simulink library "DAEMOT_Lib"  (R2019b)
settings: Solver=ode45  StartTime=0.0  StopTime=10.0  FixedStep=0.1  RelTol=1e-3
undefined symbols (not defined in the file or in its folder): Controller, CP, Ctrl, Ctrl_Fcn, Elec1, f, F2, Fluid, lag1, Mission, Moody, PropellerProp, rev_comms_sink
libraries: $bdroot x200, instrumentlib x21, simulink x5, dspsigops x2
(part 4 of 13)

== system DAEMOT_Lib/Support Functions ==
  Data Manager : Subsystem  mask{null=0}
      mask init:
      | set_param(gcb, 'LinkStatus', 'inactive')    % disable the library link
      settings: OpenFcn=data_manager
      mask Display: str ='Data Manager\n(Double click to select variables for output)'; fprintf(str)
  Data_Sink : Subsystem  LoadFcn=|  InitFcn=|  mask(Data Sink){}
      LoadFcn=|
      | h      = get_param(gcb,'handle');   % Get block handle                           
      | hblock = get(h);     % Parse out handles structure
      | 
      | str = [hblock.Path(numel(bdroot)+2:end), hblock.Name];
      | str(~ismember(str,['A':'Z' 'a':'z' '0':'9' '_'])) = '';                     
      | set_param([gcb, '/global_data_goto'],'GotoTag',['gdata_',str]);
      |                                
      |                                                                                  
      | clear h hblock str
      InitFcn=|
      | h      = get_param(gcb,'handle');   % Get block handle                           
      | hblock = get(h);     % Parse out handles structure
      | 
      | str = [hblock.Path(numel(bdroot)+2:end), hblock.Name];
      | str(~ismember(str,['A':'Z' 'a':'z' '0':'9' '_'])) = '';                     
      | set_param([gcb, '/global_data_goto'],'GotoTag',['gdata_',str]);
      |                                
      |                                                                                  
      | clear h hblock str
      mask help:
      | Input to this block should be a bus signal with named signals.
      |
      | Bus signals sent to this block will be read by the Data Manager.
      | The Data Manager will handle the global routing of signals.
      |
      | This block should be placed under the mask of components.
      settings: CopyFcn=|
      | h      = get_param(gcb,'handle');   % Get block handle
      | hblock = get(h);     % Parse out handles structure
      | 
      | str = [hblock.Path(numel(bdroot)+2:end), hblock.Name];
      | str(~ismember(str,['A':'Z' 'a':'z' '0':'9' '_'])) = '';
      | set_param([gcb, '/global_data_goto'],'GotoTag',['gdata_',str]);
      | 
      | 
      | clear h hblock str
      settings: NameChangeFcn=|
      | h      = get_param(gcb,'handle');   % Get block handle
      | hblock = get(h);     % Parse out handles structure
      | 
      | str = [hblock.Path(numel(bdroot)+2:end), hblock.Name];
      | str(~ismember(str,['A':'Z' 'a':'z' '0':'9' '_'])) = '';
      | set_param([gcb, '/global_data_goto'],'GotoTag',['gdata_',str]);
      | 
      | 
      | clear h hblock str
      mask Display: text(0.25,0.5,'Data Sink')
  Generic Graph Model : Subsystem  mask{G_NAME=Elec1, MODE=DAE Graph}
      mask prompts: G_NAME "Graph Name"; MODE "Graph Type"
      mask init:
      | %%%%% update the variant subsystem %%%%%%%%%%%%%
      | simulationStatus =  get_param(bdroot,'SimulationStatus');
      | choice = get_param(gcb,'MODE');
      | vssBlk = [gcb, '/Variant Subsystem'];
      | oldVariant = get_param(gcb,'OverrideUsingVariant');
      | if strcmp(choice,'Dynamic Graph')   
      |     set_param(vssBlk, 'OverrideUsingVariant', 'Dynamic_Graph');
      | else  
      |     set_param(vssBlk, 'OverrideUsingVariant', 'DAE_Graph');
      | end
      | 
      | %%%%%%% load in graph for property lookups %%%%%%%%%
      | GRAPH_NAME = get_param(gcb,'G_NAME');
      | 
      | Graph = evalin('base',GRAPH_NAME);
      | 
      | h      = get_param(gcb,'handle');   % Get block handle
      | blk    = gcb;
      | hblock = get(h);     % Parse out handles structure
      | 
      | blk = [gcb,'/Variant Subsystem/',choice]; 
      | 
      | if Graph.Nu == 0
      |     Nu = 1;
      | else
      |     Nu = Graph.Nu;
      | end
      | 
      | if Graph.Nsv == 0
      |     Nsv = 1;
      | else
      |     Nsv = Graph.Nsv;
      | end
      | 
      | %%%%%%%%% 1D Property Lookups %%%%%%%%%%%%%%%%%%%%%%%%%%%%%%%%%%%%
      | % delete extra blocks
      | temp = get_param([blk,'/mux_1D'],'Inputs');
      | try % check if previous operation had zero 1-D lookups
      |     get_param([blk,'/map_1D_1'],'Table');
      |     flag = 1; %if we find a lookup table, set flag high
      | catch
      |     flag = 0; %if previous operation had zero 1-D lookups, set flag low
      | end
      | 
      | if Graph.ND1_map == 0 %if there are zero property lookups, make sure the mux is of size 1
      |     set_param([blk,'/mux_1D'],'Inputs','1')
      | else
      |     set_param([blk,'/mux_1D'],'Inputs',num2str(Graph.ND1_map))
      | end
      | % delete extra blocks and lines
      | for i = Graph.ND1_map+1:str2num(temp)
      |     try
      |         delete_block([blk,'/select_1D_',num2str(i)])
      |         delete_block([blk,'/map_1D_',num2str(i)])
      |         delete_block([blk,'/mod_1D_',num2str(i)])
      |         delete_unconnected_lines(blk)
      |     catch
      |     end
      | end
      | 
      | if flag == 0 %modifier to make sure 1st lookup is added if previous graph had zero lookups
      |     temp = num2str((str2num(temp)-1));
      | end
      | 
      | %re-label existing blocks
      | if Graph.ND1_map ~= 0
      |     for i = 1:str2num(temp)     
      |         set_param([blk,'/select_1D_',num2str(i)],'InputPortWidth',[GRAPH_NAME,'.Nv+',num2str(Nsv),'+',num2str(Nu)])
      |         if Graph.Props.D1_map{2,i} == 2
      |             set_param([blk,'/select_1D_',num2str(i)],'Indices',char(horzcat(GRAPH_NAME,'.Nv+',num2str(Nsv),'+Elec.Props.D1_map{1,',num2str(i),'}')))
      |         else
      |             set_param([blk,'/select_1D_',num2str(i)],'Indices',char(horzcat(GRAPH_NAME,'.Props.D1_map{1,',num2str(i),'}')))
      |         end
      |         set_param([blk,'/map_1D_',num2str(i)],'BreakpointsForDimension1',char(horzcat(GRAPH_NAME,'.Props.D1_map{3,',num2str(i),'}')))
      |         set_param([blk,'/map_1D_',num2str(i)],'Table',char(horzcat(GRAPH_NAME,'.Props.D1_map{4,',num2str(i),'}')))
      |         if Graph.Props.D1_map{6,i} == 2
      |             set_param([blk,'/mod_1D_',num2str(i)],'Operator','reciprocal')
      |         else
      |             set_param([blk,'/mod_1D_',num2str(i)],'Operator','transpose')
      |         end
      |     end
      | end
      | 
      | 
      | % add blocks
      | if Graph.ND1_map ~= 0
      |     for i = str2num(temp)+1:Graph.ND1_map
      |         add_block('simulink/Signal Routing/Selector',        [blk,'/select_1D_',num2str(i)],    'Position',[1355 16+i*80 1355+40 16+i*80+38]);
      |         add_block('simulink/Lookup Tables/1-D Lookup Table', [blk,'/map_1D_',num2str(i)],    'Position',[1435 3+i*80 1435+65 3+i*80+64]);
      |         add_block('simulink/Math Operations/Math Function', [blk,'/mod_1D_',num2str(i)],    'Position',[1545 20+i*80 1545+30 20+i*80+30]);
      |         
      |         set_param([blk,'/select_1D_',num2str(i)],'InputPortWidth',[GRAPH_NAME,'.Nv+',num2str(Nsv),'+',num2str(Nu)])
      |         if Graph.Props.D1_map{2,i} == 2
      |             set_param([blk,'/select_1D_',num2str(i)],'Indices',char(horzcat(GRAPH_NAME,'.Nv+',num2str(Nsv),'+Elec.Props.D1_map{1,',num2str(i),'}')))
      |         else
      |             set_param([blk,'/select_1D_',num2str(i)],'Indices',char(horzcat(GRAPH_NAME,'.Props.D1_map{1,',num2str(i),'}')))
      |         end
      |         set_param([blk,'/map_1D_',num2str(i)],'BreakpointsForDimension1',char(horzcat(GRAPH_NAME,'.Props.D1_map{3,',num2str(i),'}')))
      |         set_param([blk,'/map_1D_',num2str(i)],'Table',char(horzcat(GRAPH_NAME,'.Props.D1_map{4,',num2str(i),'}')))
      |         if Graph.Props.D1_map{6,i} == 2
      |             set_param([blk,'/mod_1D_',num2str(i)],'Operator','reciprocal')
      |         else
      |             set_param([blk,'/mod_1D_',num2str(i)],'Operator','transpose')
      |         end
      |         
      |         add_line(blk,['all_1D/1'], ['select_1D_',num2str(i),'/1'],'AutoRouting','on')
      |         add_line(blk,['select_1D_',num2str(i),'/1'], ['map_1D_',num2str(i),'/1'],'AutoRouting','on')
      |         add_line(blk,['map_1D_',num2str(i),'/1'], ['mod_1D_',num2str(i),'/1'],'AutoRouting','on')
      |         add_line(blk,['mod_1D_',num2str(i),'/1'], ['mux_1D/',num2str(i)],'AutoRouting','on')
      |     end
      | end
      | 
      | %%%%%%%%% 2D Property Lookups %%%%%%%%%%%%%%%%%%%%%%%%%%%%%%%%%%%%
      | % delete extra blocks
      | temp = get_param([blk,'/mux_2D'],'Inputs');
      | try % check if previous operation had zero 1-D lookups
      |     get_param([blk,'/map_2D_1'],'Table');
      |     flag = 1; %if we find a lookup table, set flag high
      | catch
      |     flag = 0; %if previous operation had zero 1-D lookups, set flag low
      | end
      | 
      | if Graph.ND2_map == 0 %if there are zero property lookups, make sure the mux is of size 1
      |     set_param([blk,'/mux_2D'],'Inputs','1')
      | else
      |     set_param([blk,'/mux_2D'],'Inputs',num2str(Graph.ND2_map))
      | end
      | % delete extra blocks and lines
      | for i = Graph.ND2_map+1:str2num(temp)
      |     try
      |         delete_block([blk,'/select_2D_',num2str(i)])
      |         delete_block([blk,'/demux_2D_',num2str(i)])
      |         delete_block([blk,'/map_2D_',num2str(i)])
      |         delete_block([blk,'/mod_2D_',num2str(i)])
      |         delete_unconnected_lines(blk)
      |     catch
      |     end
      | end
      | 
      | if flag == 0 %modifier to make sure 1st lookup is added if previous graph had zero lookups
      |     temp = num2str((str2num(temp)-1));
      | end
      | 
      | %re-label existing blocks
      | % add blocks
      | if Graph.ND2_map ~= 0
      |     for i = 1:str2num(temp)
      |         
      |         set_param([blk,'/select_2D_',num2str(i)],'InputPortWidth',[GRAPH_NAME,'.Nv+',num2str(Nsv),'+',num2str(Nu)])
      |         if Graph.Props.D2_map{2,i} == 2           
      |             set_param([blk,'/select_2D_',num2str(i)],'Indices',char(horzcat('[',GRAPH_NAME,'.Props.D2_map{1,',num2str(i),'}(1), ',GRAPH_NAME,'.Nv+',num2str(Nsv),'+',GRAPH_NAME,'.Props.D2_map{1,',num2str(i),'}(2)]')))
      |         else
      |             set_param([blk,'/select_2D_',num2str(i)],'Indices',char(horzcat(GRAPH_NAME,'.Props.D2_map{1,',num2str(i),'}')))           
      |         end
      |         %         set_param([blk,'/select_2D_',num2str(i)],'IndexParamArray',{char(horzcat('Elec.Props.D2_map{1,',num2str(i),'}'))})
      |         set_param([blk,'/map_2D_',num2str(i)],'BreakpointsForDimension1',char(horzcat(GRAPH_NAME,'.Props.D2_map{3,',num2str(i),'}{1,1}')))
      |         set_param([blk,'/map_2D_',num2str(i)],'BreakpointsForDimension2',char(horzcat(GRAPH_NAME,'.Props.D2_map{3,',num2str(i),'}{2,1}')))
      |         set_param([blk,'/map_2D_',num2str(i)],'Table',char(horzcat(GRAPH_NAME,'.Props.D2_map{4,',num2str(i),horzcat('}',''''))))
      |         if Graph.Props.D2_map{6,i} == 1
      |             set_param([blk,'/mod_2D_',num2str(i)],'Operator','transpose')
      |         else
      |             set_param([blk,'/mod_2D_',num2str(i)],'Operator','reciprocal')
      |         end
      |      
      |     end
      | end
      | 
      | % add blocks
      | if Graph.ND2_map ~= 0
      |     for i = str2num(temp)+1:Graph.ND2_map
      |         add_block('simulink/Signal Routing/Selector',        [blk,'/select_2D_',num2str(i)],    'Position',[1925 16+i*80 1925+40 16+i*80+38]);
      |         add_block('simulink/Signal Routing/Demux',           [blk,'/demux_2D_',num2str(i)],    'Position',[2020 15+i*80 2020+5 15+i*80+40]);
      |         add_block('simulink/Lookup Tables/2-D Lookup Table', [blk,'/map_2D_',num2str(i)],    'Position',[2085 15+i*80 2085+40 15+i*80+40]);
      |         add_block('simulink/Math Operations/Math Function',  [blk,'/mod_2D_',num2str(i)],    'Position',[2180 20+i*80 2180+30 20+i*80+30]);
      |         
      |         set_param([blk,'/select_2D_',num2str(i)],'InputPortWidth',[GRAPH_NAME,'.Nv+',num2str(Nsv),'+',num2str(Nu)])
      |         if Graph.Props.D2_map{2,i} == 2           
      |             set_param([blk,'/select_2D_',num2str(i)],'Indices',char(horzcat('[',GRAPH_NAME,'.Props.D2_map{1,',num2str(i),'}(1), ',GRAPH_NAME,'.Nv+',num2str(Nsv),'+',GRAPH_NAME,'.Props.D2_map{1,',num2str(i),'}(2)]')))
      |         else
      |             set_param([blk,'/select_2D_',num2str(i)],'Indices',char(horzcat(GRAPH_NAME,'.Props.D2_map{1,',num2str(i),'}')))           
      |         end
      |         %         set_param([blk,'/select_2D_',num2str(i)],'IndexParamArray',{char(horzcat('Elec.Props.D2_map{1,',num2str(i),'}'))})
      |         set_param([blk,'/map_2D_',num2str(i)],'BreakpointsForDimension1',char(horzcat(GRAPH_NAME,'.Props.D2_map{3,',num2str(i),'}{1,1}')))
      |         set_param([blk,'/map_2D_',num2str(i)],'BreakpointsForDimension2',char(horzcat(GRAPH_NAME,'.Props.D2_map{3,',num2str(i),'}{2,1}')))
      |         set_param([blk,'/map_2D_',num2str(i)],'Table',char(horzcat(GRAPH_NAME,'.Props.D2_map{4,',num2str(i),horzcat('}',''''))))
      |         if Graph.Props.D2_map{6,i} == 1
      |             set_param([blk,'/mod_2D_',num2str(i)],'Operator','transpose')
      |         else
      |             set_param([blk,'/mod_2D_',num2str(i)],'Operator','reciprocal')
      |         end
      |         
      |         add_line(blk,['all_2D/1'], ['select_2D_',num2str(i),'/1'],'AutoRouting','on')
      |         add_line(blk,['select_2D_',num2str(i),'/1'], ['demux_2D_',num2str(i),'/1'],'AutoRouting','on')
      |         add_line(blk,['demux_2D_',num2str(i),'/1'], ['map_2D_',num2str(i),'/1'],'AutoRouting','on')
      |         add_line(blk,['demux_2D_',num2str(i),'/2'], ['map_2D_',num2str(i),'/2'],'AutoRouting','on')
      |         add_line(blk,['map_2D_',num2str(i),'/1'], ['mod_2D_',num2str(i),'/1'],'AutoRouting','on')
      |         add_line(blk,['mod_2D_',num2str(i),'/1'], ['mux_2D/',num2str(i)],'AutoRouting','on')
      |     end
      | end
      | 
      | %%%% old iterations of code. I've updated this to delete and replace all
      | %%%% blocks at each update of the block
      | 
      | % % % % %%%%%%%%% 1D Property Lookups %%%%%%%%%%%%%%%%%%%%%%%%%%%%%%%%%%%%
      | % % % % % delete extra blocks
      | % % % % temp = get_param([blk,'/mux_1D'],'Inputs');
      | % % % % try % check if previous operation had zero 1-D lookups
      | % % % %     get_param([blk,'/map_1D_1'],'Table');
      | % % % %     flag = 1; %if we find a lookup table, set flag high
      | % % % % catch
      | % % % %     flag = 0; %if previous operation had zero 1-D lookups, set flag low
      | % % % % end
      | % % % % 
      | % % % % if Elec.Nu == 0
      | % % % %     Nu = 1;
      | % % % % else
      | % % % %     Nu = Elec.Nu;
      | % % % % end
      | % % % % 
      | % % % % if Elec.Nsv == 0
      | % % % %     Nsv = 1;
      | % % % % else
      | % % % %     Nsv = Elec.Nsv;
      | % % % % end
      | % % % % 
      | % % % % if Elec.ND1_map == 0 %if there are zero property lookups, make sure the mux is of size 1
      | % % % %     set_param([blk,'/mux_1D'],'Inputs','1')
      | % % % % else
      | % % % %     set_param([blk,'/mux_1D'],'Inputs',num2str(Elec.ND1_map))
      | % % % % end
      | % % % % % delete extra blocks and lines
      | % % % % for i = Elec.ND1_map+1:str2num(temp)
      | % % % %     try
      | % % % %         delete_block([blk,'/select_1D_',num2str(i)])
      | % % % %         delete_block([blk,'/map_1D_',num2str(i)])
      | % % % %         delete_block([blk,'/mod_1D_',num2str(i)])
      | % % % %         delete_unconnected_lines(blk)
      | % % % %     catch
      | % % % %     end
      | % % % % end
      | % % % % 
      | % % % % if flag == 0 %modifier to make sure 1st lookup is added if previous graph had zero lookups
      | % % % %     temp = num2str((str2num(temp)-1))
      | % % % % end
      | % % % % 
      | % % % % % add blocks
      | % % % % if Elec.ND1_map ~= 0
      | % % % %     for i = str2num(temp)+1:Elec.ND1_map
      | % % % %         add_block('simulink/Signal Routing/Selector',        [blk,'/select_1D_',num2str(i)],    'Position',[1355 16+i*80 1355+40 16+i*80+38]);
      | % % % %         add_block('simulink/Lookup Tables/1-D Lookup Table', [blk,'/map_1D_',num2str(i)],    'Position',[1435 3+i*80 1435+65 3+i*80+64]);
      | % % % %         add_block('simulink/Math Operations/Math Function', [blk,'/mod_1D_',num2str(i)],    'Position',[1545 20+i*80 1545+30 20+i*80+30]);
      | % % % %         
      | % % % %         set_param([blk,'/select_1D_',num2str(i)],'InputPortWidth',['Elec.Nv+',num2str(Nsv),'+',num2str(Nu)])
      | % % % %         if Elec.Props.D1_map{2,i} == 2
      | % % % %             set_param([blk,'/select_1D_',num2str(i)],'Indices',char(horzcat('Elec.Nv+',num2str(Nsv),'+Elec.Props.D1_map{1,',num2str(i),'}')))
      | % % % %         else
      | % % % %             set_param([blk,'/select_1D_',num2str(i)],'Indices',char(horzcat('Elec.Props.D1_map{1,',num2str(i),'}')))
      | % % % %         end
      | % % % %         set_param([blk,'/map_1D_',num2str(i)],'BreakpointsForDimension1',char(horzcat('Elec.Props.D1_map{3,',num2str(i),'}')))
      | % % % %         set_param([blk,'/map_1D_',num2str(i)],'Table',char(horzcat('Elec.Props.D1_map{4,',num2str(i),'}')))
      | % % % %         if Elec.Props.D1_map{6,i} == 2
      | % % % %             set_param([blk,'/mod_1D_',num2str(i)],'Operator','reciprocal')
      | % % % %         else
      | % % % %             set_param([blk,'/mod_1D_',num2str(i)],'Operator','transpose')
      | % % % %         end
      | % % % %         
      | % % % %         add_line(blk,['all_1D/1'], ['select_1D_',num2str(i),'/1'],'AutoRouting','on')
      | % % % %         add_line(blk,['select_1D_',num2str(i),'/1'], ['map_1D_',num2str(i),'/1'],'AutoRouting','on')
      | % % % %         add_line(blk,['map_1D_',num2str(i),'/1'], ['mod_1D_',num2str(i),'/1'],'AutoRouting','on')
      | % % % %         add_line(blk,['mod_1D_',num2str(i),'/1'], ['mux_1D/',num2str(i)],'AutoRouting','on')
      | % % % %     end
      | % % % % end
      | 
      | % % % % %%%%%%%%% 2D Property Lookups %%%%%%%%%%%%%%%%%%%%%%%%%%%%%%%%%%%%
      | % % % % % delete extra blocks
      | % % % % temp = get_param([blk,'/mux_2D'],'Inputs');
      | % % % % try % check if previous operation had zero 1-D lookups
      | % % % %     get_param([blk,'/map_2D_1'],'Table');
      | % % % %     flag = 1; %if we find a lookup table, set flag high
      | % % % % catch
      | % % % %     flag = 0; %if previous operation had zero 1-D lookups, set flag low
      | % % % % end
      | % % % % 
      | % % % % if Elec.ND2_map == 0 %if there are zero property lookups, make sure the mux is of size 1
      | % % % %     set_param([blk,'/mux_2D'],'Inputs','1')
      | % % % % else
      | % % % %     set_param([blk,'/mux_2D'],'Inputs',num2str(Elec.ND2_map))
      | % % % % end
      | % % % % % delete extra blocks and lines
      | % % % % for i = Elec.ND2_map+1:str2num(temp)
      | % % % %     try
      | % % % %         delete_block([blk,'/select_2D_',num2str(i)])
      | % % % %         delete_block([blk,'/demux_2D_',num2str(i)])
      | % % % %         delete_block([blk,'/map_2D_',num2str(i)])
      | % % % %         delete_block([blk,'/mod_2D_',num2str(i)])
      | % % % %         delete_unconnected_lines(blk)
      | % % % %     catch
      | % % % %     end
      | % % % % end
      | % % % % 
      | % % % % if flag == 0 %modifier to make sure 1st lookup is added if previous graph had zero lookups
      | % % % %     temp = num2str((str2num(temp)-1))
      | % % % % end
      | % % % % 
      | % % % % % add blocks
      | % % % % if Elec.ND2_map ~= 0
      | % % % %     for i = str2num(temp)+1:Elec.ND2_map
      | % % % %         add_block('simulink/Signal Routing/Selector',        [blk,'/select_2D_',num2str(i)],    'Position',[1925 16+i*80 1925+40 16+i*80+38]);
      | % % % %         add_block('simulink/Signal Routing/Demux',           [blk,'/demux_2D_',num2str(i)],    'Position',[2020 15+i*80 2020+5 15+i*80+40]);
      | % % % %         add_block('simulink/Lookup Tables/2-D Lookup Table', [blk,'/map_2D_',num2str(i)],    'Position',[2085 15+i*80 2085+40 15+i*80+40]);
      | % % % %         add_block('simulink/Math Operations/Math Function',  [blk,'/mod_2D_',num2str(i)],    'Position',[2180 20+i*80 2180+30 20+i*80+30]);
      | % % % %         
      | % % % %         set_param([blk,'/select_2D_',num2str(i)],'InputPortWidth',['Elec.Nv+',num2str(Nsv),'+',num2str(Nu)])
      | % % % %         if Elec.Props.D2_map{2,i} == 2           
      | % % % %             set_param([blk,'/select_2D_',num2str(i)],'Indices',char(horzcat('[Elec.Props.D2_map{1,',num2str(i),'}(1), Elec.Nv+',num2str(Nsv),'+Elec.Props.D2_map{1,',num2str(i),'}(2)]')))
      | % % % %         else
      | % % % %             set_param([blk,'/select_2D_',num2str(i)],'Indices',char(horzcat('Elec.Props.D2_map{1,',num2str(i),'}')))           
      | % % % %         end
      | % % % %         %         set_param([blk,'/select_2D_',num2str(i)],'IndexParamArray',{char(horzcat('Elec.Props.D2_map{1,',num2str(i),'}'))})
      | % % % %         set_param([blk,'/map_2D_',num2str(i)],'BreakpointsForDimension1',char(horzcat('Elec.Props.D2_map{3,',num2str(i),'}{1,1}')))
      | % % % %         set_param([blk,'/map_2D_',num2str(i)],'BreakpointsForDimension2',char(horzcat('Elec.Props.D2_map{3,',num2str(i),'}{2,1}')))
      | % % % %         set_param([blk,'/map_2D_',num2str(i)],'Table',char(horzcat('Elec.Props.D2_map{4,',num2str(i),horzcat('}',''''))))
      | % % % %         if Elec.Props.D2_map{6,i} == 1
      | % % % %             set_param([blk,'/mod_2D_',num2str(i)],'Operator','transpose')
      | % % % %         else
      | % % % %             set_param([blk,'/mod_2D_',num2str(i)],'Operator','reciprocal')
      | % % % %         end
      | % % % %         
      | % % % %         add_line(blk,['all_2D/1'], ['select_2D_',num2str(i),'/1'],'AutoRouting','on')
      | % % % %         add_line(blk,['select_2D_',num2str(i),'/1'], ['demux_2D_',num2str(i),'/1'],'AutoRouting','on')
      | % % % %         add_line(blk,['demux_2D_',num2str(i),'/1'], ['map_2D_',num2str(i),'/1'],'AutoRouting','on')
      | % % % %         add_line(blk,['demux_2D_',num2str(i),'/2'], ['map_2D_',num2str(i),'/2'],'AutoRouting','on')
      | % % % %         add_line(blk,['map_2D_',num2str(i),'/1'], ['mod_2D_',num2str(i),'/1'],'AutoRouting','on')
      | % % % %         add_line(blk,['mod_2D_',num2str(i),'/1'], ['mux_2D/',num2str(i)],'AutoRouting','on')
      | % % % %     end
      | % % % % end
      mask TypeOptions MODE: Dynamic Graph | DAE Graph
      mask Display:
      | G_NAME = get_param(gcb,'G_NAME');
      | 
      | text(0.5,0.95,['{\bf' G_NAME '}'],'TexMode','on','horizontalAlignment', 'center');
      | 
      | 
      | port_label('input',1,'Inputs [ordered]')
      | port_label('input',2,'Source Vertex [ordered]')
      | port_label('input',3,'Source Edge [ordered]')
      | 
      | port_label('output',1,'States')
      | port_label('output',2,'Power Flows')
  Generic Sink : Subsystem  mask(Effort Sink (Torque)){Stype=Voltage Sink, const=on, value=0}
      mask prompts: Stype "Sink Type"; const "Constant Value?"; value "Voltage [V]"
      mask help: Used to create a effot sink.
      mask init: same as DAEMOT_Lib/Electrical/Effort Sink
      settings: CopyFcn=|
      | h      = get_param(gcb,'handle');   % Get block handle
      | blk    = gcb;
      | 
      | set_param(blk, 'LinkStatus', 'inactive')
      | clear h
      | clear blk
      mask TypeOptions Stype: Voltage Sink | Current Sink | Angular Speed Sink | Torque Sink | Temperature Sink | Heat Flow Sink | Pressure Sink | Mass Flow Sink
      mask Callback Stype:
      | mp     = get_param(gcb,'MaskPrompts');
      | h      = get_param(gcb,'handle');   % Get block handle
      | blk    = gcb;
      | hblock = get(h);     % Parse out handles structure
      | 
      | switch get_param(gcb,'Stype')
      |     case 'Voltage Sink'
      |         mp{3} = 'Voltage [V]';
      |     case 'Current Sink'
      |         mp{3} = 'Current [A]';
      |     case 'Angular Speed Sink'
      |         mp{3} = 'Speed [rad/s]';
      |     case 'Torque Sink'
      |         mp{3} = 'Torque [Nm]';
      |     case 'Temperature Sink'
      |         mp{3} = 'Temperature [C]';
      |     case 'Heat Flow Sink'
      |         mp{3} = 'Heat Flow [kW]';
      |     case 'Pressure Sink'
      |         mp{3} = 'Pressure [kPa]';
      |     case 'Mass Flow Sink'
      |         mp{3} = 'Mass Flow [kg/s]';
      | end
      | set_param(gcb,'MaskPrompts',mp);
      | 
      | clear mp h blk hblock
      mask Callback const:
      | en = get_param(gcb,'MaskVisibilities');
      | h      = get_param(gcb,'handle');   % Get block handle
      | blk    = gcb;
      | hblock = get(h);     % Parse out handles structure
      | 
      | switch get_param(gcb,'const')
      |     case 'on'
      |         en{3} = 'on';
      | %         delete_block([blk,'/In1'])
      | 
      |     case 'off'
      |         en{3} = 'off';
      | %         add_block('simulink/Ports & Subsystems/In1',   [blk,'/In1'],'Position',[130    -7   160     7]);         % adding inport
      | 
      | end
      | set_param(gcb,'MaskVisibilities',en);
      | 
      | % hblock.MaskPrompts{3} = 'hello';
      | clear en h blk hblock
      mask Display:
      | text(0.5,0.90,['{\bf',get_param(gcb,'Stype'),'}'],'TexMode','on','horizontalAlignment', 'center')
      | % text(0.5,0.1,['{(T)(end)}'],'TexMode','on','horizontalAlignment', 'center')
      | 
      | type = get_param(gcb,'Stype');
      | switch type
      |         case 'Voltage Sink'
      |             nm = 'Voltage [V]';
      |             id = '(V)';
      |             un = 'V';
      |         case 'Current Sink'
      |             nm = 'Current [A]';
      |             id = '(----)';
      |             un = 'A';
      |         case 'Angular Speed Sink'
      |             nm = 'Speed [rad/s]';
      |             id = '(----)';
      |             un = 'rad/s';
      |         case 'Torque Sink'
      |             nm = 'Torque [Nm]';
      |             id = '(\tau)';
      |             un = 'Nm';
      |         case 'Temperature Sink'
      |             nm = 'Temperature [C]';
      |             id = '(T)';
      |             un = 'C';
      |         case 'Heat Flow Sink'
      |             nm = 'Heat Flow [kW]';
      |             id = '(----)';
      |             un = 'kW';
      |         case 'Pressure Sink'
      |             nm = 'Pressure [kPa]';
      |             id = '(P)';
      |             un = 'kPa';
      |         case 'Mass Flow Sink'
      |             nm = 'Mass Flow [kg/s]';
      |             id = '(----)';
      |             un = 'kg/s';
      | end
      | 
      | if strcmp(get_param(gcb,'const'),'on')
      |     text(0.75,0.500,['{\bf',get_param(gcb,'Value'),un,'}'],'TexMode','on','horizontalAlignment', 'center')
      | else
      |     port_label('input',2,sprintf(['Sink ',nm]));
      | end
      | 
      | 
      | port_label('input',1,'Sink');
      | text(0.5,0.175,['{',id,' (end)}'],'TexMode','on','horizontalAlignment', 'center');
  Generic Source : Subsystem  mask(Effort Source (Voltage)){Stype=Voltage Source, const=on, value=0}
      mask prompts: Stype "Source Type"; const "Constant Value?"; value "Voltage [V]"
      mask help: Used to create an effort source.
      mask init:
      | h      = get_param(gcb,'handle');   % Get block handle
      | blk    = gcb;
      | hblock = get(h);     % Parse out handles structure
      | type = get_param(gcb,'Stype');
      |         
      | switch type
      |     case 'Voltage Source'
      |         up = 'current';
      |         dw = 'voltage';
      |     case 'Current Source'
      |         dw = 'current';
      |         up = 'voltage';
      |     case 'Angular Speed Source'
      |         up = 'torque';
      |         dw = 'aspeed';
      |     case 'Torque Source'
      |         dw = 'torque';
      |         up = 'aspeed';
      |     case 'Temperature Source'
      |         up = 'Q_kW';
      |         dw = 'Temp';
      |     case 'Heat Flow Source'
      |         dw = 'Q_kW';
      |         up = 'Temp';
      |     case 'Pressure Source'
      |         up = 'mdot_kgps';
      |         mid= 'T_C';
      |         dw = 'P_kPa';
      |     case 'Mass Flow Source'
      |         up = 'mdot_kgps';
      |         mid= 'T_C';
      |         dw = 'P_kPa';
      | end
      | 
      | if (((type(1) == 'P') || (type(1) == 'M')) && (const == 1)) %if constant input (user defined in mask) and need temperature input
      |     
      |     try add_block('simulink/Ports & Subsystems/In1', [blk,'/In2'], 'Position', [200,230,230,245]) %make temperature input
      |         set_param([blk, '/b1'],'Inputs','3');
      |         add_line(blk,'In2/1','b1/3','AutoRouting','on');
      |             
      |         p = get_param([blk,'/In2'],'PortHandles');
      |         l = get_param(p.Outport,'Line');
      |         set_param(l,'Name',mid);
      |     end 
      |     
      |     try delete_block([blk,'/In1'])
      |         delete_unconnected_lines(blk);
      |         
      |         fprintf ("option 1\n");        
      |         
      |         add_block('simulink/Sources/Constant',   [blk,'/val'], 'Position', [200,148,230,162]);
      |         add_line(blk,'val/1','b1/2','AutoRouting','on');
      |         set_param([blk,'/val'],'Value','value');
      |         
      |         p = get_param([blk,'/Constant'],'PortHandles');
      |         l = get_param(p.Outport,'Line');
      |         set_param(l,'Name',up);
      | 
      |         p = get_param([blk,'/val'],'PortHandles');
      |         l = get_param(p.Outport,'Line');
      |         set_param(l,'Name',dw);
      |         
      |     end
      |     p = get_param([blk,'/Constant'],'PortHandles');
      |     l = get_param(p.Outport,'Line');
      | 
      |     if (strcmp(get_param(l,'name'),up)) %If it didn't work and l's name doesn't match what it should, set them again.
      |     else
      |         set_param(l,'Name',up);
      |         
      |         fprintf ("failed strcmp \n");
      |                 
      |         p = get_param([blk,'/val'],'PortHandles');
      |         l = get_param(p.Outport,'Line');
      |         set_param(l,'Name',dw);
      |             
      |         p = get_param([blk,'/In2'],'PortHandles');
      |         l = get_param(p.Outport,'Line');
      |         set_param(l,'Name',mid);
      |     end
      |     
      | elseif ((type(1) == 'P') || (type(1) == 'M')) %if need input port (not user defined in mask) and also need temperature input
      |     
      |     try add_block('simulink/Ports & Subsystems/In1', [blk,'/In2'], 'Position', [200,230,230,245]) %make temperature input
      |         set_param([blk, '/b1'],'Inputs','3');
      |         add_line(blk,'In2/1','b1/3','AutoRouting','on');
      | 
      |         p = get_param([blk,'/In2'],'PortHandles');
      |         l = get_param(p.Outport,'Line');
      |         set_param(l,'Name',mid);
      |     end
      |     
      |     try delete_block([blk,'/val'])
      |         delete_unconnected_lines(blk);
      |         
      |         fprintf ("option 2\n");      
      |         
      |         add_block('simulink/Ports & Subsystems/In1', [blk,'/In1'], 'Position', [200,148,230,162]);
      |         add_line(blk,'In1/1','b1/2','AutoRouting','on');
      |         
      |         p = get_param([blk,'/Constant'],'PortHandles');
      |         l = get_param(p.Outport,'Line');
      |         set_param(l,'Name',up);
      | 
      |         p = get_param([blk,'/In1'],'PortHandles');
      |         l = get_param(p.Outport,'Line');
      |         set_param(l,'Name',dw);
      |         
      |     end
      |     
      |     p = get_param([blk,'/Constant'],'PortHandles');
      |     l = get_param(p.Outport,'Line');
      |     if (strcmp(get_param(l,'name'),up)) %If it didn't work and l's name doesn't match what it should, set them again.
      |     else
      |         set_param(l,'Name',up);
      |         
      |         fprintf ("failed strcmp \n");
      |         
      |         p = get_param([blk,'/In1'],'PortHandles');
      |         l = get_param(p.Outport,'Line');
      |         set_param(l,'Name',dw);
      | 
      |         p = get_param([blk,'/In2'],'PortHandles');
      |         l = get_param(p.Outport,'Line');
      |         set_param(l,'Name',mid);
      |     end
      |     
      | elseif (const == 1) %if constant, user-defined input, but does not need a temperature input port
      |     try delete_block([blk,'/In2']) %delete temperature input
      |         delete_unconnected_lines(blk);
      |         
      |         set_param([blk, '/b1'],'Inputs','2');
      |         fprintf ("delete in2 \n");
      |     end
      |     
      |     try delete_block([blk,'/In1'])
      |         delete_unconnected_lines(blk);
      |         
      |         fprintf ("option 3\n");
      |         
      |         add_block('simulink/Sources/Constant',   [blk,'/val'], 'Position', [200,198,230,212]);
      |         add_line(blk,'val/1','b1/2','AutoRouting','on');
      |         set_param([blk,'/val'],'Value','value');
      |         
      |         p = get_param([blk,'/Constant'],'PortHandles');
      |         l = get_param(p.Outport,'Line');
      |         set_param(l,'Name',up);
      |         
      |         p = get_param([blk,'/val'],'PortHandles');
      |         l = get_param(p.Outport,'Line');
      |         set_param(l,'Name',dw);
      |     end
      |     
      |     p = get_param([blk,'/Constant'],'PortHandles');
      |     l = get_param(p.Outport,'Line');
      |     if (strcmp(get_param(l,'name'),up))
      |     else
      |         set_param(l,'Name',up);
      |         
      |         fprintf ("failed strcmp \n");
      |                 
      |         p = get_param([blk,'/val'],'PortHandles');
      |         l = get_param(p.Outport,'Line');
      |         set_param(l,'Name',dw);
      |     end
      |     
      | else %if need an input port for the input, but not for temperature
      |     try delete_block([blk,'/In2']) %delete temperature input
      |         delete_unconnected_lines(blk);
      |         
      |         set_param([blk, '/b1'],'Inputs','2');
      |         fprintf ("deleted in2 \n");
      |     end    
      |         
      |     try delete_block([blk,'/val'])
      |         delete_unconnected_lines(blk);
      |         
      |         fprintf ("option 4\n");
      |         
      |         add_block('simulink/Ports & Subsystems/In1',   [blk,'/In1'], 'Position', [200,198,230,212]);
      |         add_line(blk,'In1/1','b1/2','AutoRouting','on');
      |         
      |         p = get_param([blk,'/Constant'],'PortHandles');
      |         l = get_param(p.Outport,'Line');
      |         set_param(l,'Name',up);
      | 
      |         p = get_param([blk,'/In1'],'PortHandles');
      |         l = get_param(p.Outport,'Line');
      |         set_param(l,'Name',dw);
      |     end
      |     
      |     p = get_param([blk,'/Constant'],'PortHandles');
      |     l = get_param(p.Outport,'Line');
      |     if (strcmp(get_param(l,'name'),up))
      |     else
      |         set_param(l,'Name',up);
      |         fprintf ("failed strcmp \n");
      |         p = get_param([blk,'/In1'],'PortHandles');
      |         l = get_param(p.Outport,'Line');
      |         set_param(l,'Name',dw);
      |     end
      |     
      | end
      | 
      | 
      | %if const == 1;
      | %    try delete_block([blk,'/In1'])
      | %        delete_unconnected_lines(blk);
      | %        add_block('simulink/Sources/Constant',   [blk,'/val'], 'Position', [200,198,230,212]);
      | %        add_line(blk,'val/1','b1/2','AutoRouting','on');
      | %        set_param([blk,'/val'],'Value','value');
      | 
      | %        p = get_param([blk,'/Constant'],'PortHandles');
      | %        l = get_param(p.Outport,'Line');
      | %        set_param(l,'Name',up);
      |         
      | %        p = get_param([blk,'/val'],'PortHandles');
      | %        l = get_param(p.Outport,'Line');
      | %        set_param(l,'Name',dw);
      | %    end
      | %    p = get_param([blk,'/Constant'],'PortHandles');
      | %    l = get_param(p.Outport,'Line');
      | %    if strcmp(get_param(l,'name'),up)
      | %    else
      | %       set_param(l,'Name',up);
      |         
      | %        p = get_param([blk,'/val'],'PortHandles');
      | %        l = get_param(p.Outport,'Line');
      | %        set_param(l,'Name',dw);
      | %    end
      |      
      | %%     delete_unconnected_lines(blk)
      | %else
      | %    try delete_block([blk,'/val'])
      | %        delete_unconnected_lines(blk);
      | %        add_block('simulink/Ports & Subsystems/In1',   [blk,'/In1'], 'Position', [200,198,230,212]);
      | %        add_line(blk,'In1/1','b1/2','AutoRouting','on');
      |         
      | %        p = get_param([blk,'/Constant'],'PortHandles');
      | %        l = get_param(p.Outport,'Line');
      | %        set_param(l,'Name',up);
      | 
      | %        p = get_param([blk,'/In1'],'PortHandles');
      | %        l = get_param(p.Outport,'Line');
      | %        set_param(l,'Name',dw);
      | %    end
      | %    p = get_param([blk,'/Constant'],'PortHandles');
      | %    l = get_param(p.Outport,'Line');
      | %    if strcmp(get_param(l,'name'),up)
      | %    else
      | %        set_param(l,'Name',up);
      |         
      | %        p = get_param([blk,'/In1'],'PortHandles');
      | %        l = get_param(p.Outport,'Line');
      | %        set_param(l,'Name',dw);
      | %    end
      | %end
      | 
      | clear h blk hblock type
      settings: CopyFcn=|
      | h      = get_param(gcb,'handle');   % Get block handle
      | blk    = gcb;
      | 
      | set_param(blk, 'LinkStatus', 'inactive')
      | clear h
      | clear blk
      mask TypeOptions Stype: Voltage Source | Current Source | Angular Speed Source | Torque Source | Temperature Source | Heat Flow Source | Pressure Source | Mass Flow Source
      mask Callback Stype:
      | mp     = get_param(gcb,'MaskPrompts');
      | h      = get_param(gcb,'handle');   % Get block handle
      | blk    = gcb;
      | hblock = get(h);     % Parse out handles structure
      | 
      | switch get_param(gcb,'Stype')
      |     case 'Voltage Source'
      |         mp{3} = 'Voltage [V]';
      |     case 'Current Source'
      |         mp{3} = 'Current [A]';
      |     case 'Angular Speed Source'
      |         mp{3} = 'Speed [rad/s]';
      |     case 'Torque Source'
      |         mp{3} = 'Torque [Nm]';
      |     case 'Temperature Source'
      |         mp{3} = 'Temperature [C]';
      |     case 'Heat Flow Source'
      |         mp{3} = 'Heat Flow [kW]';
      |     case 'Pressure Source'
      |         mp{3} = 'Pressure [kPa]';
      |     case 'Mass Flow Source'
      |         mp{3} = 'Mass Flow [kg/s]';
      | end
      | set_param(gcb,'MaskPrompts',mp);
      | 
      | clear mp h blk hblock
      mask Callback const:
      | en = get_param(gcb,'MaskVisibilities');
      | h      = get_param(gcb,'handle');   % Get block handle
      | blk    = gcb;
      | hblock = get(h);     % Parse out handles structure
      | 
      | switch get_param(gcb,'const')
      |     case 'on'
      |         en{3} = 'on';
      | %         delete_block([blk,'/In1'])
      | 
      |     case 'off'
      |         en{3} = 'off';
      | %         add_block('simulink/Ports & Subsystems/In1',   [blk,'/In1'],'Position',[130    -7   160     7]);         % adding inport
      | 
      | end
      | set_param(gcb,'MaskVisibilities',en);
      | 
      | % hblock.MaskPrompts{3} = 'hello';
      | clear en h blk hblock
      mask Display:
      | text(0.5,0.900,['{\bf',get_param(gcb,'Stype'),'}'],'TexMode','on','horizontalAlignment', 'center')
      | 
      | type = get_param(gcb,'Stype');
      | switch type
      |     case 'Voltage Source'
      |         nm = 'Voltage [V]';
      |         id = '(V)*';
      |         un = 'V';
      |     case 'Current Source'
      |         nm = 'Current [A]';
      |         id = '(----)';
      |         un = 'A';
      |     case 'Angular Speed Source'
      |         nm = 'Speed [rad/s]';
      |         id = '(----)';
      |         un = 'rad/s';
      |     case 'Torque Source'
      |         nm = 'Torque [Nm]';
      |         id = '(\tau)*';
      |         un = 'Nm';
      |     case 'Temperature Source'
      |         nm = 'Temperature [C]';
      |         id = '(T)';
      |         un = 'C';
      |     case 'Heat Flow Source'
      |         nm = 'Heat Flow [kW]';
      |         id = '(----)';
      |         un = 'kW';
      |     case 'Pressure Source'
      |         nm = 'Pressure [kPa]';
      |         id = '(P)';
      |         un = 'kPa';
      |     case 'Mass Flow Source'
      |         nm = 'Mass Flow [kg/s]';
      |         id = '(----)';
      |         un = 'kg/s';
      | end
      | 
      | if strcmp(get_param(gcb,'const'),'on')
      |     text(0.35,0.500,['{\bf',get_param(gcb,'Value'),un,'}'],'TexMode','on','horizontalAlignment', 'center')
      | else
      |     port_label('input',1,sprintf(['Source \n',nm]))
      | end
      | port_label('output',1,'Source')
      | text(0.5,0.175,['{(start) ',id,'}'],'TexMode','on','horizontalAlignment', 'center')
      | 
      | switch type
      |     case 'Pressure Source'
      |         if strcmp(get_param(gcb,'const'),'off')
      |             port_label('input',2,sprintf(['Source\nTemp. [C]']))
      |         else
      |             port_label('input',1,sprintf(['Source\nTemp. [C]']))
      | 
      |         end
      |     case 'Mass Flow Source'
      |         if strcmp(get_param(gcb,'const'),'off')
      |             port_label('input',2,sprintf(['Source\nTemp. [C]']))
      |         else
      |             port_label('input',1,sprintf(['Source\nTemp. [C]']))
      | 
      |         end
      | end
  Mission Preview : Subsystem  TreatAsAtomicUnit=on  SystemSampleTime=DT  mask(Preview of Signals){timeseries=Mission, DT=1, hor=10}
      mask prompts: timeseries "Signal (timeseries object):"; DT "Update rate (seconds)"; hor "Prediction horizon (Np)"
      mask help: Signal should be formatted as a MATLAB timeseries object.
      mask Display:
      | h      = get_param(gcb,'handle');   % Get block handle
      | blk    = gcb;
      | hblock = get(h);     % Parse out handles structure
      | 
      | text(0.5,0.75,'Preview of:','horizontalAlignment', 'center')
      | text(0.5,0.35,hblock.timeseries,'horizontalAlignment', 'center')
  Real-Time Communication : Subsystem
      mask Display: image(imread('Analog_Flow.jpg'))
  Sink : Subsystem  LoadFcn=rev_comms_sink();  InitFcn=rev_comms_sink();  mask(Sink){}
      mask help: Used for sending data to the upstream component.
      settings: CopyFcn=rev_comms_sink();  NameChangeFcn=rev_comms_sink();
      mask Display: text(0.25,0.5,'Sink')
  Source : Subsystem  mask(Source){}
      mask help: Used for receiving data from the downstream component.
      mask init:
      | n_src = gcb;
      | n_src = str2num(n_src(end));
      | try
      |     rev_comms_source(n_src);
      | catch
      | 
      | end
      mask Display: text(0.25,0.5,'Source')
  "Unit Conversion " : Subsystem  mask(Unit conversion){mass=off, frommass=Grams, tomass=Pounds-Mass, dens=off, fromdens=Pounds-Mass, perdens=Cubic Feet, todens=Kilograms, toperdens=Cubic Meters, energy=off, fromenergy=Joules, toenergy=Joules, power=off, frompower=Kilowatts, topower=Watts, force=off, fromforce=Newtons, toforce=Newtons, temp=on, fromtemp=Fahrenheit, totemp=Celcius, pres=off, frompres=psia, topres=psia, length=off, fromlength=Millimeters, tolength=Millimeters, area=off, fromarea=Square Centimeters, toarea=Square Centimeters, vol=off, fromvol=Milliliters, tovol=Milliliters, vel=off, fromlen=Millimeters, fromtime=Millisecond, tolen=Millimeters, totime=Millisecond, flow_rate=off, fromflowvol=Milliliters, fromflvoltime=Millisecond, toflowvol=Milliliters, toflvoltime=Millisecond, mfr=off, frommfr=Grams, frommfrtime=Millisecond, tomfr=Grams, tomfrtime=Millisecond}
      mask prompts: frommass "From :"; tomass "To :"; dens "Density"; fromdens "From :"; perdens "per"; todens "To :"; toperdens "per"; fromenergy "From :"; toenergy "To :"; frompower "From :"; topower "To :"; fromforce "From :"; toforce "To :"; temp "Temperature"; fromtemp "From :"; totemp "To :"; pres "Pressure"; frompres "From :"; topres "To :"; fromlength "From :"; tolength "To :"; fromarea "From :"; toarea "To :"; vol "Volume"; fromvol "From :"; tovol "To :"; vel "Velocity"; fromlen "From :........."; fromtime "per"; tolen "To :.........."; totime "per"; flow_rate "Volume Flow Rate"; fromflowvol "From :........."; fromflvoltime "per"; toflowvol "To :.........."; toflvoltime "per"; mfr "Mass Flow Rate"; frommfr "From :........."; frommfrtime "per"; tomfr "To :.........."; tomfrtime "per"
      mask help:
      | Convert units of:
      |
      | Mass, density, energy, power, force, temperature, pressure, length, area, volume, velocity, and flow rate
      mask init:
      | %set_param(gcb, 'linkstatus', 'inactive')
      | 
      | %cellarr = get_param(gcb,'MaskVisibilities') ;
      | %ind = [1 4 9 12 15 18 21 24 27 30 33 38 43] ;
      | 
      | %cellarr(1:length(cellarr)) = {'off'} ;
      | %cellarr(ind) = {'on'};
      | %set_param(blk,'MaskVisibilities',cellarr) ;
      mask Callback mass:
      | blk = gcb ;
      | value = get_param(blk,'mass') ;
      | cellarr = get_param(blk,'MaskVisibilities') ;
      | ind = [1 4 9 12 15 18 21 24 27 30 33 38 43] ;
      | if strcmp(value,'on')
      |     cellarr(ind) = {'off'} ; cellarr(1:3) = {'on'} ;
      |     value1 = get_param(blk,'frommass') ;
      |     value2 = get_param(blk,'tomass') ;
      |     if strcmp(get_param(blk,'mass'),'on') ;
      |         switch value1
      |             case 'Grams'
      |                 name1 = 'gr' ;
      |                 fcn1  = 'u(1)*.001' ;
      |             case 'Kilograms'
      |                 name1 = 'kg' ;
      |                 fcn1  = 'u(1)' ;
      |             case 'Ounces'
      |                 name1 = 'oz' ;
      |                 fcn1  = 'u(1)*.45359237/16' ;
      |             case 'Pounds-Mass'
      |                 name1 = 'lbm' ;
      |                 fcn1  = 'u(1)*.45359237' ;
      |             case 'Slugs'
      |                 name1 = 'slg' ;
      |                 fcn1  = 'u(1)*14.5939029' ;
      |         end
      |         switch value2
      |             case 'Grams'
      |                 name2 = 'gr' ;
      |                 fcn2  = '/.001' ;
      |             case 'Kilograms'
      |                 name2 = 'kg' ;
      |                 fcn2  = '' ;
      |             case 'Ounces'
      |                 name2 = 'oz' ;
      |                 fcn2  = '/.45359237*16' ;
      |             case 'Pounds-Mass'
      |                 name2 = 'lbm' ;
      |                 fcn2  = '/.45359237' ;
      |             case 'Slugs'
      |                 name2 = 'slg' ;
      |                 fcn2  = '/14.5939029' ;
      |         end
      |         expr = [fcn1 fcn2] ;
      |         %set_param(blk,'func',func) ;
      |         set_param([blk '/conv_fcn'],'expr',expr) ;
      |         str1 = ['% this block of text is updated via dialog callbacks'];
      |         str2 = [char(39) 'horizontalAlignment' char(39) ',' char(39) 'center' char(39) ',' char(39) 'texmode' char(39) ',' char(39) 'on' char(39)] ;
      |         name = [char(39) name1 ' to ' name2 char(39)] ;
      |         str = sprintf('%s\ntext(.5,.5,%s,%s)',str1,name,str2) ;
      |         set_param(blk,'MaskDisplay',str) ;
      |     end
      |     clear value1 value2 expr name1 name2 name fcn1 fcn2 str1 str2 str
      | else
      |     cellarr(2:3) = {'off'} ; val = get_param(blk,'MaskValues') ;
      |     for i=1:length(ind)
      |         a = findstr(val{ind(i)},'on') ;
      |         b(i) = isempty(a) ;
      |     end
      |     if isempty(find(b==0)) ;
      |         cellarr(ind) = {'on'} ;
      |     end
      | end
      | set_param(blk,'MaskVisibilities',cellarr) ;
      | clear blk value cellarr ind a b val i
      mask TypeOptions frommass: Grams | Kilograms | Ounces | Pounds-Mass | Slugs
      mask Callback frommass:
      | blk = gcb ;
      | value1 = get_param(blk,'frommass') ;
      | value2 = get_param(blk,'tomass') ;
      | if strcmp(get_param(blk,'mass'),'on') ;
      |     switch value1
      |         case 'Grams'
      |             name1 = 'gr' ;
      |             fcn1  = 'u(1)*.001' ;
      |         case 'Kilograms'
      |             name1 = 'kg' ;
      |             fcn1  = 'u(1)' ;
      |         case 'Ounces'
      |             name1 = 'oz' ;
      |             fcn1  = 'u(1)*.45359237/16' ;
      |         case 'Pounds-Mass'
      |             name1 = 'lbm' ;
      |             fcn1  = 'u(1)*.45359237' ;
      |         case 'Slugs'
      |             name1 = 'slg' ;
      |             fcn1  = 'u(1)*14.5939029' ;
      |     end
      |     switch value2
      |         case 'Grams'
      |             name2 = 'gr' ;
      |             fcn2  = '/.001' ;
      |         case 'Kilograms'
      |             name2 = 'kg' ;
      |             fcn2  = '' ;
      |         case 'Ounces'
      |             name2 = 'oz' ;
      |             fcn2  = '/.45359237*16' ;
      |         case 'Pounds-Mass'
      |             name2 = 'lbm' ;
      |             fcn2  = '/.45359237' ;
      |         case 'Slugs'
      |             name2 = 'slg' ;
      |             fcn2  = '/14.5939029' ;
      |     end
      |     expr = [fcn1 fcn2] ;
      |     %set_param(blk,'func',func) ;
      |     set_param([blk '/conv_fcn'],'expr',expr) ;
      |     str1 = ['% this block of text is updated via dialog callbacks'];
      |         str2 = [char(39) 'horizontalAlignment' char(39) ',' char(39) 'center' char(39) ',' char(39) 'texmode' char(39) ',' char(39) 'on' char(39)] ;
      |     name = [char(39) name1 ' to ' name2 char(39)] ;
      |     str = sprintf('%s\ntext(.5,.5,%s,%s)',str1,name,str2) ;
      |     set_param(blk,'MaskDisplay',str) ;
      | end
      |     clear blk value1 value2 expr name1 name2 name fcn1 fcn2 str1 str2 str
      mask TypeOptions tomass: Grams | Kilograms | Ounces | Pounds-Mass | Slugs
      mask Callback tomass:
      | blk = gcb ;
      | value1 = get_param(blk,'frommass') ;
      | value2 = get_param(blk,'tomass') ;
      | if strcmp(get_param(blk,'mass'),'on') ;
      |     switch value1
      |         case 'Grams'
      |             name1 = 'gr' ;
      |             fcn1  = 'u(1)*.001' ;
      |         case 'Kilograms'
      |             name1 = 'kg' ;
      |             fcn1  = 'u(1)' ;
      |         case 'Ounces'
      |             name1 = 'oz' ;
      |             fcn1  = 'u(1)*.45359237/16' ;
      |         case 'Pounds-Mass'
      |             name1 = 'lbm' ;
      |             fcn1  = 'u(1)*.45359237' ;
      |         case 'Slugs'
      |             name1 = 'slg' ;
      |             fcn1  = 'u(1)*14.5939029' ;
      |     end
      |     switch value2
      |         case 'Grams'
      |             name2 = 'gr' ;
      |             fcn2  = '/.001' ;
      |         case 'Kilograms'
      |             name2 = 'kg' ;
      |             fcn2  = '' ;
      |         case 'Ounces'
      |             name2 = 'oz' ;
      |             fcn2  = '/.45359237*16' ;
      |         case 'Pounds-Mass'
      |             name2 = 'lbm' ;
      |             fcn2  = '/.45359237' ;
      |         case 'Slugs'
      |             name2 = 'slg' ;
      |             fcn2  = '/14.5939029' ;
      |     end
      |     expr = [fcn1 fcn2] ;
      |     %set_param(blk,'func',func) ;
      |     set_param([blk '/conv_fcn'],'expr',expr) ;
      |     str1 = ['% this block of text is updated via dialog callbacks'];
      |         str2 = [char(39) 'horizontalAlignment' char(39) ',' char(39) 'center' char(39) ',' char(39) 'texmode' char(39) ',' char(39) 'on' char(39)] ;
      |     name = [char(39) name1 ' to ' name2 char(39)] ;
      |     str = sprintf('%s\ntext(.5,.5,%s,%s)',str1,name,str2) ;
      |     set_param(blk,'MaskDisplay',str) ;
      | end
      |     clear blk value1 value2 expr name1 name2 name fcn1 fcn2 str1 str2 str
      mask Callback dens:
      | blk = gcb ;
      | value = get_param(blk,'dens') ;
      | cellarr = get_param(blk,'MaskVisibilities');
      | ind = [1 4 9 12 15 18 21 24 27 30 33 38 43] ;
      | if strcmp(value,'on')
      |     cellarr(ind) = {'off'} ; cellarr(4:8) = {'on'} ;
      |     value1 = get_param(blk,'fromdens') ;
      |     value2 = get_param(blk,'perdens') ;
      |     value3 = get_param(blk,'todens') ;
      |     value4 = get_param(blk,'toperdens') ;
      |     if strcmp(get_param(blk,'dens'),'on')
      |         switch value1
      |             case 'Grams'
      |                 name1 = 'g/' ;
      |                 fcn1  = 'u(1)*.001' ;
      |             case 'Kilograms'
      |                 name1 = 'kg/' ;
      |                 fcn1  = 'u(1)' ;
      |             case 'Ounces'
      |                 name1 = 'oz/' ;
      |                 fcn1  = 'u(1)*.45359237/16' ;
      |             case 'Pounds-Mass'
      |                 name1 = 'lbm/' ;
      |                 fcn1  = 'u(1)*.45359237' ;
      |             case 'Slugs'
      |                 name1 = 'slg/' ;
      |                 fcn1  = 'u(1)*14.5939';
      |         end
      |         switch value2
      |             case 'Milliliters'
      |                 name2 = 'mL' ;
      |                 fcn2  = '/(1e-6)' ;
      |             case 'Liters'
      |                 name2 = 'L' ;
      |                 fcn2  = '/.001' ;
      |             case 'Cubic Centimeters'
      |                 name2 = 'cm^3' ;
      |                 fcn2  = '/(1e-6)' ;
      |             case 'Cubic Meters'
      |                 name2 = 'm^3' ;
      |                 fcn2  = '' ;
      |             case 'Ounces'
      |                 name2 = 'oz' ;
      |                 fcn2  = '/(2.95735e-5)' ;
      |             case 'Gallons'
      |                 name2 = 'gal' ;
      |                 fcn2  = '/.0037854' ;
      |             case 'Cubic Inches'
      |                 name2 = 'in^3' ;
      |                 fcn2  = '/(1.6387e-5)' ;
      |             case 'Cubic Feet'
      |                 name2 = 'ft^3' ;
      |                 fcn2  = '/.02831685' ;
      |         end
      |         switch value3
      |             case 'Grams'
      |                 name3 = 'g/' ;
      |                 fcn3  = '/.001' ;
      |             case 'Kilograms'
      |                 name3 = 'kg/' ;
      |                 fcn3  = '' ;
      |             case 'Ounces'
      |                 name3 = 'oz/' ;
      |                 fcn3  = '/.45359237*16' ;
      |             case 'Pounds-Mass'
      |                 name3 = 'lbm/' ;
      |                 fcn3  = '/.45359237' ;
      |             case 'Slugs'
      |                 name3 = 'slg/' ;
      |                 fcn3  = '/14.5939';
      |         end
      |         switch value4
      |             case 'Milliliters'
      |                 name4 = 'mL' ;
      |                 fcn4  = '*(1e-6)' ;
      |             case 'Liters'
      |                 name4 = 'L' ;
      |                 fcn4  = '*.001' ;
      |             case 'Cubic Centimeters'
      |                 name4 = 'cm^3' ;
      |                 fcn4  = '*(1e-6)' ;
      |             case 'Cubic Meters'
      |                 name4 = 'm^3' ;
      |                 fcn4  = '' ;
      |             case 'Ounces'
      |                 name4 = 'oz' ;
      |                 fcn4  = '*(2.95735e-5)' ;
      |             case 'Gallons'
      |                 name4 = 'gal' ;
      |                 fcn4  = '*.0037854' ;
      |             case 'Cubic Inches'
      |                 name4 = 'in^3' ;
      |                 fcn4  = '*(1.6387e-5)' ;
      |             case 'Cubic Feet'
      |                 name4 = 'ft^3' ;
      |                 fcn4  = '*.02831685' ;
      |         end
      |         expr = [fcn1 fcn2 fcn3 fcn4] ;
      |         %set_param(blk,'func',func) ;
      |         set_param([blk '/conv_fcn'],'expr',expr) ;
      |         str1 = ['% this block of text is updated via dialog callbacks'];
      |         str2 = [char(39) 'horizontalAlignment' char(39) ',' char(39) 'center' char(39) ',' char(39) 'texmode' char(39) ',' char(39) 'on' char(39)] ;
      |         name = [char(39) name1 name2 ' to ' name3 name4 char(39)] ;
      |         str = sprintf('%s\ntext(.5,.5,%s,%s)',str1,name,str2) ;
      |         set_param(blk,'MaskDisplay',str) ;
      |     end
      |     clear value1 value2 value3 value4 expr name1 name2 name3 name4 name fcn1 fcn2 fcn3 fcn4 str1 str2 str
      | 
      | else
      |     cellarr(5:8) = {'off'} ; val = get_param(blk,'MaskValues') ;
      |     for i=1:length(ind)
      |         a = findstr(val{ind(i)},'on') ;
      |         b(i) = isempty(a) ;
      |     end
      |     if isempty(find(b==0)) ;
      |         cellarr(ind) = {'on'} ;
      |     end
      | end
      | set_param(blk,'MaskVisibilities',cellarr) ;
      | clear blk value cellarr ind a b val i
      mask TypeOptions fromdens: Grams | Kilograms | Ounces | Pounds-Mass | Slugs
      mask Callback fromdens:
      | blk = gcb ;
      | value1 = get_param(blk,'fromdens') ;
      | value2 = get_param(blk,'perdens') ;
      | value3 = get_param(blk,'todens') ;
      | value4 = get_param(blk,'toperdens') ;
      | if strcmp(get_param(blk,'dens'),'on')
      |     switch value1
      |         case 'Grams'
      |             name1 = 'g/' ;
      |             fcn1  = 'u(1)*.001' ;
      |         case 'Kilograms'
      |             name1 = 'kg/' ;
      |             fcn1  = 'u(1)' ;
      |         case 'Ounces'
      |             name1 = 'oz/' ;
      |             fcn1  = 'u(1)*.45359237/16' ;
      |         case 'Pounds-Mass'
      |             name1 = 'lbm/' ;
      |             fcn1  = 'u(1)*.45359237' ;
      |         case 'Slugs'
      |             name1 = 'slg/' ;
      |             fcn1  = 'u(1)*14.5939';
      |     end
      |     switch value2
      |         case 'Milliliters'
      |             name2 = 'mL' ;
      |             fcn2  = '/(1e-6)' ;
      |         case 'Liters'
      |             name2 = 'L' ;
      |             fcn2  = '/.001' ;
      |         case 'Cubic Centimeters'
      |             name2 = 'cm^3' ;
      |             fcn2  = '/(1e-6)' ;
      |         case 'Cubic Meters'
      |             name2 = 'm^3' ;
      |             fcn2  = '' ;
      |         case 'Ounces'
      |             name2 = 'oz' ;
      |             fcn2  = '/(2.95735e-5)' ;
      |         case 'Gallons'
      |             name2 = 'gal' ;
      |             fcn2  = '/.0037854' ;
      |         case 'Cubic Inches'
      |             name2 = 'in^3' ;
      |             fcn2  = '/(1.6387e-5)' ;
      |         case 'Cubic Feet'
      |             name2 = 'ft^3' ;
      |             fcn2  = '/.02831685' ;
      |     end
      |     switch value3
      |         case 'Grams'
      |             name3 = 'g/' ;
      |             fcn3  = '/.001' ;
      |         case 'Kilograms'
      |             name3 = 'kg/' ;
      |             fcn3  = '' ;
      |         case 'Ounces'
      |             name3 = 'oz/' ;
      |             fcn3  = '/.45359237*16' ;
      |         case 'Pounds-Mass'
      |             name3 = 'lbm/' ;
      |             fcn3  = '/.45359237' ;
      |         case 'Slugs'
      |             name3 = 'slg/' ;
      |             fcn3  = '/14.5939';
      |     end
      |     switch value4
      |         case 'Milliliters'
      |             name4 = 'mL' ;
      |             fcn4  = '*(1e-6)' ;
      |         case 'Liters'
      |             name4 = 'L' ;
      |             fcn4  = '*.001' ;
      |         case 'Cubic Centimeters'
      |             name4 = 'cm^3' ;
      |             fcn4  = '*(1e-6)' ;
      |         case 'Cubic Meters'
      |             name4 = 'm^3' ;
      |             fcn4  = '' ;
      |         case 'Ounces'
      |             name4 = 'oz' ;
      |             fcn4  = '*(2.95735e-5)' ;
      |         case 'Gallons'
      |             name4 = 'gal' ;
      |             fcn4  = '*.0037854' ;
      |         case 'Cubic Inches'
      |             name4 = 'in^3' ;
      |             fcn4  = '*(1.6387e-5)' ;
      |         case 'Cubic Feet'
      |             name4 = 'ft^3' ;
      |             fcn4  = '*.02831685' ;
      |     end
      |     expr = [fcn1 fcn2 fcn3 fcn4] ;
      |     %set_param(blk,'func',func) ;
      |     set_param([blk '/conv_fcn'],'expr',expr) ;
      |     str1 = ['% this block of text is updated via dialog callbacks'];
      |     str2 = [char(39) 'horizontalAlignment' char(39) ',' char(39) 'center' char(39) ',' char(39) 'texmode' char(39) ',' char(39) 'on' char(39)] ;
      |     name = [char(39) name1 name2 ' to ' name3 name4 char(39)] ;
      |     str = sprintf('%s\ntext(.5,.5,%s,%s)',str1,name,str2) ;
      |     set_param(blk,'MaskDisplay',str) ;
      | end
      | clear blk value1 value2 value3 value4 expr name1 name2 name3 name4 name fcn1 fcn2 fcn3 fcn4 str1 str2 str
      mask TypeOptions perdens: Milliliters | Liters | Cubic Centimeters | Cubic Meters | Ounces | Gallons | Cubic Inches | Cubic Feet
      mask Callback perdens:
      | blk = gcb ;
      | value1 = get_param(blk,'fromdens') ;
      | value2 = get_param(blk,'perdens') ;
      | value3 = get_param(blk,'todens') ;
      | value4 = get_param(blk,'toperdens') ;
      | if strcmp(get_param(blk,'dens'),'on')
      |     switch value1
      |         case 'Grams'
      |             name1 = 'g/' ;
      |             fcn1  = 'u(1)*.001' ;
      |         case 'Kilograms'
      |             name1 = 'kg/' ;
      |             fcn1  = 'u(1)' ;
      |         case 'Ounces'
      |             name1 = 'oz/' ;
      |             fcn1  = 'u(1)*.45359237/16' ;
      |         case 'Pounds-Mass'
      |             name1 = 'lbm/' ;
      |             fcn1  = 'u(1)*.45359237' ;
      |         case 'Slugs'
      |             name1 = 'slg/' ;
      |             fcn1  = 'u(1)*14.5939';
      |     end
      |     switch value2
      |         case 'Milliliters'
      |             name2 = 'mL' ;
      |             fcn2  = '/(1e-6)' ;
      |         case 'Liters'
      |             name2 = 'L' ;
      |             fcn2  = '/.001' ;
      |         case 'Cubic Centimeters'
      |             name2 = 'cm^3' ;
      |             fcn2  = '/(1e-6)' ;
      |         case 'Cubic Meters'
      |             name2 = 'm^3' ;
      |             fcn2  = '' ;
      |         case 'Ounces'
      |             name2 = 'oz' ;
      |             fcn2  = '/(2.95735e-5)' ;
      |         case 'Gallons'
      |             name2 = 'gal' ;
      |             fcn2  = '/.0037854' ;
      |         case 'Cubic Inches'
      |             name2 = 'in^3' ;
      |             fcn2  = '/(1.6387e-5)' ;
      |         case 'Cubic Feet'
      |             name2 = 'ft^3' ;
      |             fcn2  = '/.02831685' ;
      |     end
      |     switch value3
      |         case 'Grams'
      |             name3 = 'g/' ;
      |             fcn3  = '/.001' ;
      |         case 'Kilograms'
      |             name3 = 'kg/' ;
      |             fcn3  = '' ;
      |         case 'Ounces'
      |             name3 = 'oz/' ;
      |             fcn3  = '/.45359237*16' ;
      |         case 'Pounds-Mass'
      |             name3 = 'lbm/' ;
      |             fcn3  = '/.45359237' ;
      |         case 'Slugs'
      |             name3 = 'slg/' ;
      |             fcn3  = '/14.5939';
      |     end
      |     switch value4
      |         case 'Milliliters'
      |             name4 = 'mL' ;
      |             fcn4  = '*(1e-6)' ;
      |         case 'Liters'
      |             name4 = 'L' ;
      |             fcn4  = '*.001' ;
      |         case 'Cubic Centimeters'
      |             name4 = 'cm^3' ;
      |             fcn4  = '*(1e-6)' ;
      |         case 'Cubic Meters'
      |             name4 = 'm^3' ;
      |             fcn4  = '' ;
      |         case 'Ounces'
      |             name4 = 'oz' ;
      |             fcn4  = '*(2.95735e-5)' ;
      |         case 'Gallons'
      |             name4 = 'gal' ;
      |             fcn4  = '*.0037854' ;
      |         case 'Cubic Inches'
      |             name4 = 'in^3' ;
      |             fcn4  = '*(1.6387e-5)' ;
      |         case 'Cubic Feet'
      |             name4 = 'ft^3' ;
      |             fcn4  = '*.02831685' ;
      |     end
      |     expr = [fcn1 fcn2 fcn3 fcn4] ;
      |     %set_param(blk,'func',func) ;
      |     set_param([blk '/conv_fcn'],'expr',expr) ;
      |     str1 = ['% this block of text is updated via dialog callbacks'];
      |     str2 = [char(39) 'horizontalAlignment' char(39) ',' char(39) 'center' char(39) ',' char(39) 'texmode' char(39) ',' char(39) 'on' char(39)] ;
      |     name = [char(39) name1 name2 ' to ' name3 name4 char(39)] ;
      |     str = sprintf('%s\ntext(.5,.5,%s,%s)',str1,name,str2) ;
      |     set_param(blk,'MaskDisplay',str) ;
      | end
      | clear blk value1 value2 value3 value4 expr name1 name2 name3 name4 name fcn1 fcn2 fcn3 fcn4 str1 str2 str
      mask TypeOptions todens: Grams | Kilograms | Ounces | Pounds-Mass | Slugs
      mask Callback todens:
      | blk = gcb ;
      | value1 = get_param(blk,'fromdens') ;
      | value2 = get_param(blk,'perdens') ;
      | value3 = get_param(blk,'todens') ;
      | value4 = get_param(blk,'toperdens') ;
      | if strcmp(get_param(blk,'dens'),'on')
      |     switch value1
      |         case 'Grams'
      |             name1 = 'g/' ;
      |             fcn1  = 'u(1)*.001' ;
      |         case 'Kilograms'
      |             name1 = 'kg/' ;
      |             fcn1  = 'u(1)' ;
      |         case 'Ounces'
      |             name1 = 'oz/' ;
      |             fcn1  = 'u(1)*.45359237/16' ;
      |         case 'Pounds-Mass'
      |             name1 = 'lbm/' ;
      |             fcn1  = 'u(1)*.45359237' ;
      |         case 'Slugs'
      |             name1 = 'slg/' ;
      |             fcn1  = 'u(1)*14.5939';
      |     end
      |     switch value2
      |         case 'Milliliters'
      |             name2 = 'mL' ;
      |             fcn2  = '/(1e-6)' ;
      |         case 'Liters'
      |             name2 = 'L' ;
      |             fcn2  = '/.001' ;
      |         case 'Cubic Centimeters'
      |             name2 = 'cm^3';
      |             fcn2  = '/(1e-6)' ;
      |         case 'Cubic Meters'
      |             name2 = 'm^3' ;
      |             fcn2  = '' ;
      |         case 'Ounces'
      |             name2 = 'oz' ;
      |             fcn2  = '/(2.95735e-5)' ;
      |         case 'Gallons'
      |             name2 = 'gal' ;
      |             fcn2  = '/.0037854' ;
      |         case 'Cubic Inches'
      |             name2 = 'in^3' ;
      |             fcn2  = '/(1.6387e-5)' ;
      |         case 'Cubic Feet'
      |             name2 = 'ft^3' ;
      |             fcn2  = '/.02831685' ;
      |     end
      |     switch value3
      |         case 'Grams'
      |             name3 = 'g/' ;
      |             fcn3  = '/.001' ;
      |         case 'Kilograms'
      |             name3 = 'kg/' ;
      |             fcn3  = '' ;
      |         case 'Ounces'
      |             name3 = 'oz/' ;
      |             fcn3  = '/.45359237*16' ;
      |         case 'Pounds-Mass'
      |             name3 = 'lbm/' ;
      |             fcn3  = '/.45359237' ;
      |         case 'Slugs'
      |             name3 = 'slg/' ;
      |             fcn3  = '/14.5939';
      |     end
      |     switch value4
      |         case 'Milliliters'
      |             name4 = 'mL' ;
      |             fcn4  = '*(1e-6)' ;
      |         case 'Liters'
      |             name4 = 'L' ;
      |             fcn4  = '*.001' ;
      |         case 'Cubic Centimeters'
      |             name4 = 'cm^3' ;
      |             fcn4  = '*(1e-6)' ;
      |         case 'Cubic Meters'
      |             name4 = 'm^3' ;
      |             fcn4  = '' ;
      |         case 'Ounces'
      |             name4 = 'oz' ;
      |             fcn4  = '*(2.95735e-5)' ;
      |         case 'Gallons'
      |             name4 = 'gal' ;
      |             fcn4  = '*.0037854' ;
      |         case 'Cubic Inches'
      |             name4 = 'in^3' ;
      |             fcn4  = '*(1.6387e-5)' ;
      |         case 'Cubic Feet'
      |             name4 = 'ft^3' ;
      |             fcn4  = '*.02831685' ;
      |     end
      |     expr = [fcn1 fcn2 fcn3 fcn4] ;
      |     %set_param(blk,'func',func) ;
      |     set_param([blk '/conv_fcn'],'expr',expr) ;
      |     str1 = ['% this block of text is updated via dialog callbacks'];
      |     str2 = [char(39) 'horizontalAlignment' char(39) ',' char(39) 'center' char(39) ',' char(39) 'texmode' char(39) ',' char(39) 'on' char(39)] ;
      |     name = [char(39) name1 name2 ' to ' name3 name4 char(39)] ;
      |     str = sprintf('%s\ntext(.5,.5,%s,%s)',str1,name,str2) ;
      |     set_param(blk,'MaskDisplay',str) ;
      | end
      | clear blk value1 value2 value3 value4 expr name1 name2 name3 name4 name fcn1 fcn2 fcn3 fcn4 str1 str2 str
      mask TypeOptions toperdens: Milliliters | Liters | Cubic Centimeters | Cubic Meters | Ounces | Gallons | Cubic Inches | Cubic Feet
      mask Callback toperdens:
      | blk = gcb ;
      | value1 = get_param(blk,'fromdens') ;
      | value2 = get_param(blk,'perdens') ;
      | value3 = get_param(blk,'todens') ;
      | value4 = get_param(blk,'toperdens') ;
      | if strcmp(get_param(blk,'dens'),'on')
      |     switch value1
      |         case 'Grams'
      |             name1 = 'g/' ;
      |             fcn1  = 'u(1)*.001' ;
      |         case 'Kilograms'
      |             name1 = 'kg/' ;
      |             fcn1  = 'u(1)' ;
      |         case 'Ounces'
      |             name1 = 'oz/' ;
      |             fcn1  = 'u(1)*.45359237/16' ;
      |         case 'Pounds-Mass'
      |             name1 = 'lbm/' ;
      |             fcn1  = 'u(1)*.45359237' ;
      |         case 'Slugs'
      |             name1 = 'slg/' ;
      |             fcn1  = 'u(1)*14.5939';
      |     end
      |     switch value2
      |         case 'Milliliters'
      |             name2 = 'mL' ;
      |             fcn2  = '/(1e-6)' ;
      |         case 'Liters'
      |             name2 = 'L' ;
      |             fcn2  = '/.001' ;
      |         case 'Cubic Centimeters'
      |             name2 = 'cm^3' ;
      |             fcn2  = '/(1e-6)' ;
      |         case 'Cubic Meters'
      |             name2 = 'm^3' ;
      |             fcn2  = '' ;
      |         case 'Ounces'
      |             name2 = 'oz' ;
      |             fcn2  = '/(2.95735e-5)' ;
      |         case 'Gallons'
      |             name2 = 'gal' ;
      |             fcn2  = '/.0037854' ;
      |         case 'Cubic Inches'
      |             name2 = 'in^3' ;
      |             fcn2  = '/(1.6387e-5)' ;
      |         case 'Cubic Feet'
      |             name2 = 'ft^3' ;
      |             fcn2  = '/.02831685' ;
      |     end
      |     switch value3
      |         case 'Grams'
      |             name3 = 'g/' ;
      |             fcn3  = '/.001' ;
      |         case 'Kilograms'
      |             name3 = 'kg/' ;
      |             fcn3  = '' ;
      |         case 'Ounces'
      |             name3 = 'oz/' ;
      |             fcn3  = '/.45359237*16' ;
      |         case 'Pounds-Mass'
      |             name3 = 'lbm/' ;
      |             fcn3  = '/.45359237' ;
      |         case 'Slugs'
      |             name3 = 'slg/' ;
      |             fcn3  = '/14.5939';
      |     end
      |     switch value4
      |         case 'Milliliters'
      |             name4 = 'mL' ;
      |             fcn4  = '*(1e-6)' ;
      |         case 'Liters'
      |             name4 = 'L' ;
      |             fcn4  = '*.001' ;
      |         case 'Cubic Centimeters'
      |             name4 = 'cm^3' ;
      |             fcn4  = '*(1e-6)' ;
      |         case 'Cubic Meters'
      |             name4 = 'm^3' ;
      |             fcn4  = '' ;
      |         case 'Ounces'
      |             name4 = 'oz' ;
      |             fcn4  = '*(2.95735e-5)' ;
      |         case 'Gallons'
      |             name4 = 'gal' ;
      |             fcn4  = '*.0037854' ;
      |         case 'Cubic Inches'
      |             name4 = 'in^3' ;
      |             fcn4  = '*(1.6387e-5)' ;
      |         case 'Cubic Feet'
      |             name4 = 'ft^3' ;
      |             fcn4  = '*.02831685' ;
      |     end
      |     expr = [fcn1 fcn2 fcn3 fcn4] ;
      |     %set_param(blk,'func',func) ;
      |     set_param([blk '/conv_fcn'],'expr',expr) ;
      |     str1 = ['% this block of text is updated via dialog callbacks'];
      |     str2 = [char(39) 'horizontalAlignment' char(39) ',' char(39) 'center' char(39) ',' char(39) 'texmode' char(39) ',' char(39) 'on' char(39)] ;
      |     name = [char(39) name1 name2 ' to ' name3 name4 char(39)] ;
      |     str = sprintf('%s\ntext(.5,.5,%s,%s)',str1,name,str2) ;
      |     set_param(blk,'MaskDisplay',str) ;
      | end
      | clear blk value1 value2 value3 value4 expr name1 name2 name3 name4 name fcn1 fcn2 fcn3 fcn4 str1 str2 str
      mask Callback energy:
      | blk = gcb ;
      | value = get_param(blk,'energy') ;
      | cellarr = get_param(blk,'MaskVisibilities') ;
      | ind = [1 4 9 12 15 18 21 24 27 30 33 38 43] ;
      | if strcmp(value,'on')
      |     cellarr(ind) = {'off'} ; cellarr(9:11) = {'on'} ;
      |     value1 = get_param(blk,'fromenergy') ;
      |     value2 = get_param(blk,'toenergy') ;
      |     if strcmp(get_param(blk,'energy'),'on') ;
      |         switch value1
      |             case 'Joules'
      |                 name1 = 'J' ;
      |                 fcn1  = 'u(1)' ;
      |             case 'Btu'
      |                 name1 = 'Btu' ;
      |                 fcn1  = 'u(1)*1055.05585' ;
      |             case 'Calories'
      |                 name1 = 'Cal' ;
      |                 fcn1  = 'u(1)*4.1868' ;
      |             case 'Foot-Pound(force)'
      |                 name1 = 'ft-lbf' ;
      |                 fcn1  = 'u(1)*1.355818' ;
      |             case 'Kilowatt-hour'
      |                 name1 = 'kw-hr' ;
      |                 fcn1  = 'u(1)*(3.6e6)' ;
      |         end
      |         switch value2
      |             case 'Joules'
      |                 name2 = 'J' ;
      |                 fcn2  = '' ;
      |             case 'Btu'
      |                 name2 = 'Btu' ;
      |                 fcn2  = '/1055.05585' ;
      |             case 'Calories'
      |                 name2 = 'Cal' ;
      |                 fcn2  = '/4.1868' ;
      |             case 'Foot-Pound(force)'
      |                 name2 = 'ft-lbf' ;
      |                 fcn2  = '/1.355818' ;
      |             case 'Kilowatt-hour'
      |                 name2 = 'kw-hr' ;
      |                 fcn2  = '/(3.6e6)' ;
      |         end
      |         expr = [fcn1 fcn2] ;
      |         %set_param(blk,'func',func) ;
      |         set_param([blk '/conv_fcn'],'expr',expr) ;
      |         str1 = ['% this block of text is updated via dialog callbacks'];
      |         str2 = [char(39) 'horizontalAlignment' char(39) ',' char(39) 'center' char(39) ',' char(39) 'texmode' char(39) ',' char(39) 'on' char(39)] ;
      |         name = [char(39) name1 ' to ' name2 char(39)] ;
      |         str = sprintf('%s\ntext(.5,.5,%s,%s)',str1,name,str2) ;
      |         set_param(blk,'MaskDisplay',str) ;
      |     end
      |     clear value1 value2 expr name1 name2 name fcn1 fcn2 str1 str2 str
      | else
      |     cellarr(10:11) = {'off'} ; val = get_param(blk,'MaskValues') ;
      |     for i=1:length(ind)
      |         a = findstr(val{ind(i)},'on') ;
      |         b(i) = isempty(a) ;
      |     end
      |     if isempty(find(b==0)) ;
      |         cellarr(ind) = {'on'} ;
      |     end
      | end
      | set_param(blk,'MaskVisibilities',cellarr) ;
      | clear blk value cellarr ind a b val i
      mask TypeOptions fromenergy: Joules | Btu | Calories | Foot-Pound(force) | Kilowatt-hour
      mask Callback fromenergy:
      | blk = gcb ;
      | value1 = get_param(blk,'fromenergy') ;
      | value2 = get_param(blk,'toenergy') ;
      | if strcmp(get_param(blk,'energy'),'on') ;
      |     switch value1
      |         case 'Joules'
      |             name1 = 'J' ;
      |             fcn1  = 'u(1)' ;
      |         case 'Btu'
      |             name1 = 'Btu' ;
      |             fcn1  = 'u(1)*1055.05585' ;
      |         case 'Calories'
      |             name1 = 'Cal' ;
      |             fcn1  = 'u(1)*4.1868' ;
      |         case 'Foot-Pound(force)'
      |             name1 = 'ft-lbf' ;
      |             fcn1  = 'u(1)*1.355818' ;
      |         case 'Kilowatt-hour'
      |             name1 = 'kw-hr' ;
      |             fcn1  = 'u(1)*(3.6e6)' ;
      |     end
      |     switch value2
      |         case 'Joules'
      |             name2 = 'J' ;
      |             fcn2  = '' ;
      |         case 'Btu'
      |             name2 = 'Btu' ;
      |             fcn2  = '/1055.05585' ;
      |         case 'Calories'
      |             name2 = 'Cal' ;
      |             fcn2  = '/4.1868' ;
      |         case 'Foot-Pound(force)'
      |             name2 = 'ft-lbf' ;
      |             fcn2  = '/1.355818' ;
      |         case 'Kilowatt-hour'
      |             name2 = 'kw-hr' ;
      |             fcn2  = '/(3.6e6)' ;
      |     end
      |     expr = [fcn1 fcn2] ;
      |     %set_param(blk,'func',func) ;
      |     set_param([blk '/conv_fcn'],'expr',expr) ;
      |     str1 = ['% this block of text is updated via dialog callbacks'];
      |     str2 = [char(39) 'horizontalAlignment' char(39) ',' char(39) 'center' char(39) ',' char(39) 'texmode' char(39) ',' char(39) 'on' char(39)] ;
      |     name = [char(39) name1 ' to ' name2 char(39)] ;
      |     str = sprintf('%s\ntext(.5,.5,%s,%s)',str1,name,str2) ;
      |     set_param(blk,'MaskDisplay',str) ;
      | end
      |     clear blk value1 value2 expr name1 name2 name fcn1 fcn2 str1 str2 str
      mask TypeOptions toenergy: Joules | Btu | Calories | Foot-Pound(force) | Kilowatt-hour
      mask Callback toenergy:
      | blk = gcb ;
      | value1 = get_param(blk,'fromenergy') ;
      | value2 = get_param(blk,'toenergy') ;
      | if strcmp(get_param(blk,'energy'),'on') ;
      |     switch value1
      |         case 'Joules'
      |             name1 = 'J' ;
      |             fcn1  = 'u(1)' ;
      |         case 'Btu'
      |             name1 = 'Btu' ;
      |             fcn1  = 'u(1)*1055.05585' ;
      |         case 'Calories'
      |             name1 = 'Cal' ;
      |             fcn1  = 'u(1)*4.1868' ;
      |         case 'Foot-Pound(force)'
      |             name1 = 'ft-lbf' ;
      |             fcn1  = 'u(1)*1.355818' ;
      |         case 'Kilowatt-hour'
      |             name1 = 'kw-hr' ;
      |             fcn1  = 'u(1)*(3.6e6)' ;
      |     end
      |     switch value2
      |         case 'Joules'
      |             name2 = 'J' ;
      |             fcn2  = '' ;
      |         case 'Btu'
      |             name2 = 'Btu' ;
      |             fcn2  = '/1055.05585' ;
      |         case 'Calories'
      |             name2 = 'Cal' ;
      |             fcn2  = '/4.1868' ;
      |         case 'Foot-Pound(force)'
      |             name2 = 'ft-lbf' ;
      |             fcn2  = '/1.355818' ;
      |         case 'Kilowatt-hour'
      |             name2 = 'kw-hr' ;
      |             fcn2  = '/(3.6e6)' ;
      |     end
      |     expr = [fcn1 fcn2] ;
      |     %set_param(blk,'func',func) ;
      |     set_param([blk '/conv_fcn'],'expr',expr) ;
      |     str1 = ['% this block of text is updated via dialog callbacks'];
      |     str2 = [char(39) 'horizontalAlignment' char(39) ',' char(39) 'center' char(39) ',' char(39) 'texmode' char(39) ',' char(39) 'on' char(39)] ;
      |     name = [char(39) name1 ' to ' name2 char(39)] ;
      |     str = sprintf('%s\ntext(.5,.5,%s,%s)',str1,name,str2) ;
      |     set_param(blk,'MaskDisplay',str) ;
      | end
      |     clear blk value1 value2 expr name1 name2 name fcn1 fcn2 str1 str2 str
      mask Callback power:
      | blk = gcb ;
      | value = get_param(blk,'power') ;
      | cellarr = get_param(blk,'MaskVisibilities') ;
      | ind = [1 4 9 12 15 18 21 24 27 30 33 38 43] ;
      | if strcmp(value,'on')
      |     cellarr(ind) = {'off'} ; cellarr(12:14) = {'on'} ;
      |     value1 = get_param(blk,'frompower') ;
      |     value2 = get_param(blk,'topower') ;
      |     if strcmp(get_param(blk,'power'),'on') ;
      |         switch value1
      |             case 'Watts'
      |                 name1 = 'W' ;
      |                 fcn1  = 'u(1)' ;
      |             case 'Kilowatts'
      |                 name1 = 'kW' ;
      |                 fcn1  = 'u(1)*1000' ;
      |             case 'Btu/s'
      |                 name1 = 'Btu/s' ;
      |                 fcn1  = 'u(1)*1055.056' ;
      |             case 'Btu/min'
      |                 name1 = 'Btu/min' ;
      |                 fcn1  = 'u(1)*17.584264' ;
      |             case 'Btu/hr'
      |                 name1 = 'Btu/hr' ;
      |                 fcn1  = 'u(1)*.293071' ;
      |             case 'Horsepower'
      |                 name1 = 'hp' ;
      |                 fcn1  = 'u(1)*745.69987' ;
      |         end
      |         switch value2
      |             case 'Watts'
      |                 name2 = 'W' ;
      |                 fcn2  = '' ;
      |             case 'Kilowatts'
      |                 name2 = 'kW' ;
      |                 fcn2  = '/1000' ;
      |             case 'Btu/s'
      |                 name2 = 'Btu/s' ;
      |                 fcn2  = '/1055.056' ;
      |             case 'Btu/min'
      |                 name2 = 'Btu/min' ;
      |                 fcn2  = '/17.584264' ;
      |             case 'Btu/hr'
      |                 name2 = 'Btu/hr' ;
      |                 fcn2  = '/.293071' ;
      |             case 'Horsepower'
      |                 name2 = 'hp' ;
      |                 fcn2  = '/745.69987' ;
      |         end
      |         expr = [fcn1 fcn2] ;
      |         %set_param(blk,'func',func) ;
      |         set_param([blk '/conv_fcn'],'expr',expr) ;
      |         str1 = ['% this block of text is updated via dialog callbacks'];
      |         str2 = [char(39) 'horizontalAlignment' char(39) ',' char(39) 'center' char(39) ',' char(39) 'texmode' char(39) ',' char(39) 'on' char(39)] ;
      |         name = [char(39) name1 ' to ' name2 char(39)] ;
      |         str = sprintf('%s\ntext(.5,.5,%s,%s)',str1,name,str2) ;
      |         set_param(blk,'MaskDisplay',str) ;
      |     end
      |     clear value1 value2 expr name1 name2 name fcn1 fcn2 str1 str2 str
      | else
      |     cellarr(13:14) = {'off'} ; val = get_param(blk,'MaskValues') ;
      |     for i=1:length(ind)
      |         a = findstr(val{ind(i)},'on') ;
      |         b(i) = isempty(a) ;
      |     end
      |     if isempty(find(b==0)) ;
      |         cellarr(ind) = {'on'} ;
      |     end
      | end
      | 
      | set_param(blk,'MaskVisibilities',cellarr) ;
      | clear blk value cellarr ind a b val i
      mask TypeOptions frompower: Watts | Kilowatts | Btu/s | Btu/min | Btu/hr | Horsepower
      mask Callback frompower:
      | blk = gcb ;
      | value1 = get_param(blk,'frompower') ;
      | value2 = get_param(blk,'topower') ;
      | if strcmp(get_param(blk,'power'),'on') ;
      |     switch value1
      |         case 'Watts'
      |             name1 = 'W' ;
      |             fcn1  = 'u(1)' ;
      |         case 'Kilowatts'
      |             name1 = 'kW' ;
      |             fcn1  = 'u(1)*1000' ;
      |         case 'Btu/s'
      |             name1 = 'Btu/s' ;
      |             fcn1  = 'u(1)*1055.056' ;
      |         case 'Btu/min'
      |             name1 = 'Btu/min' ;
      |             fcn1  = 'u(1)*17.584264' ;
      |         case 'Btu/hr'
      |             name1 = 'Btu/hr' ;
      |             fcn1  = 'u(1)*.293071' ;
      |         case 'Horsepower'
      |             name1 = 'hp' ;
      |             fcn1  = 'u(1)*745.69987' ;
      |     end
      |     switch value2
      |         case 'Watts'
      |             name2 = 'W' ;
      |             fcn2  = '' ;
      |         case 'Kilowatts'
      |             name2 = 'kW' ;
      |             fcn2  = '/1000' ;
      |         case 'Btu/s'
      |             name2 = 'Btu/s' ;
      |             fcn2  = '/1055.056' ;
      |         case 'Btu/min'
      |             name2 = 'Btu/min' ;
      |             fcn2  = '/17.584264' ;
      |         case 'Btu/hr'
      |             name2 = 'Btu/hr' ;
      |             fcn2  = '/.293071' ;
      |         case 'Horsepower'
      |             name2 = 'hp' ;
      |             fcn2  = '/745.69987' ;
      |     end
      |     expr = [fcn1 fcn2] ;
      |     %set_param(blk,'func',func) ;
      |     set_param([blk '/conv_fcn'],'expr',expr) ;
      |     str1 = ['% this block of text is updated via dialog callbacks'];
      |     str2 = [char(39) 'horizontalAlignment' char(39) ',' char(39) 'center' char(39) ',' char(39) 'texmode' char(39) ',' char(39) 'on' char(39)] ;
      |     name = [char(39) name1 ' to ' name2 char(39)] ;
      |     str = sprintf('%s\ntext(.5,.5,%s,%s)',str1,name,str2) ;
      |     set_param(blk,'MaskDisplay',str) ;
      | end
      |     clear blk value1 value2 expr name1 name2 name fcn1 fcn2 str1 str2 str
      mask TypeOptions topower: Watts | Kilowatts | Btu/s | Btu/min | Btu/hr | Horsepower
      mask Callback topower:
      | blk = gcb ;
      | value1 = get_param(blk,'frompower') ;
      | value2 = get_param(blk,'topower') ;
      | if strcmp(get_param(blk,'power'),'on') ;
      |     switch value1
      |         case 'Watts'
      |             name1 = 'W' ;
      |             fcn1  = 'u(1)' ;
      |         case 'Kilowatts'
      |             name1 = 'kW' ;
      |             fcn1  = 'u(1)*1000' ;
      |         case 'Btu/s'
      |             name1 = 'Btu/s' ;
      |             fcn1  = 'u(1)*1055.056' ;
      |         case 'Btu/min'
      |             name1 = 'Btu/min' ;
      |             fcn1  = 'u(1)*17.584264' ;
      |         case 'Btu/hr'
      |             name1 = 'Btu/hr' ;
      |             fcn1  = 'u(1)*.293071' ;
      |         case 'Horsepower'
      |             name1 = 'hp' ;
      |             fcn1  = 'u(1)*745.69987' ;
      |     end
      |     switch value2
      |         case 'Watts'
      |             name2 = 'W' ;
      |             fcn2  = '' ;
      |         case 'Kilowatts'
      |             name2 = 'kW' ;
      |             fcn2  = '/1000' ;
      |         case 'Btu/s'
      |             name2 = 'Btu/s' ;
      |             fcn2  = '/1055.056' ;
      |         case 'Btu/min'
      |             name2 = 'Btu/min' ;
      |             fcn2  = '/17.584264' ;
      |         case 'Btu/hr'
      |             name2 = 'Btu/hr' ;
      |             fcn2  = '/.293071' ;
      |         case 'Horsepower'
      |             name2 = 'hp' ;
      |             fcn2  = '/745.69987' ;
      |     end
      |     expr = [fcn1 fcn2] ;
      |     %set_param(blk,'func',func) ;
      |     set_param([blk '/conv_fcn'],'expr',expr) ;
      |     str1 = ['% this block of text is updated via dialog callbacks'];
      |     str2 = [char(39) 'horizontalAlignment' char(39) ',' char(39) 'center' char(39) ',' char(39) 'texmode' char(39) ',' char(39) 'on' char(39)] ;
      |     name = [char(39) name1 ' to ' name2 char(39)] ;
      |     str = sprintf('%s\ntext(.5,.5,%s,%s)',str1,name,str2) ;
      |     set_param(blk,'MaskDisplay',str) ;
      | end
      |     clear blk value1 value2 expr name1 name2 name fcn1 fcn2 str1 str2 str
      mask Callback force:
      | blk = gcb ;
      | value = get_param(blk,'force') ;
      | cellarr = get_param(blk,'MaskVisibilities') ;
      | ind = [1 4 9 12 15 18 21 24 27 30 33 38 43] ;
      | if strcmp(value,'on')
      |     cellarr(ind) = {'off'} ; cellarr(15:17) = {'on'} ;
      |     value1 = get_param(blk,'fromforce') ;
      |     value2 = get_param(blk,'toforce') ;
      |     if strcmp(get_param(blk,'force'),'on') ;
      |         switch value1
      |             case 'Newtons'
      |                 name1 = 'N' ;
      |                 fcn1  = 'u(1)' ;
      |             case 'Dyne'
      |                 name1 = 'dyne' ;
      |                 fcn1  = 'u(1)*(1e-5)' ;
      |             case 'Kilogram-Force'
      |                 name1 = 'kgf' ;
      |                 fcn1  = 'u(1)*9.80665' ;
      |             case 'Ton-Force'
      |                 name1 = 'tonf' ;
      |                 fcn1  = 'u(1)*8896.44323052' ;
      |             case 'Pound-Force'
      |                 name1 = 'lbf' ;
      |                 fcn1  = 'u(1)*4.448221615' ;
      |         end
      |         switch value2
      |             case 'Newtons'
      |                 name2 = 'N' ;
      |                 fcn2  = '' ;
      |             case 'Dyne'
      |                 name2 = 'dyne' ;
      |                 fcn2  = '/(1e-5)' ;
      |             case 'Kilogram-Force'
      |                 name2 = 'kgf' ;
      |                 fcn2  = '/9.80665' ;
      |             case 'Ton-Force'
      |                 name2 = 'tonf' ;
      |                 fcn2  = '/8896.44323052' ;
      |             case 'Pound-Force'
      |                 name2 = 'lbf' ;
      |                 fcn2  = '/4.448221615' ;
      |         end
      |         expr = [fcn1 fcn2] ;
      |         %set_param(blk,'func',func) ;
      |         set_param([blk '/conv_fcn'],'expr',expr) ;
      |         str1 = ['% this block of text is updated via dialog callbacks'];
      |         str2 = [char(39) 'horizontalAlignment' char(39) ',' char(39) 'center' char(39) ',' char(39) 'texmode' char(39) ',' char(39) 'on' char(39)] ;
      |         name = [char(39) name1 ' to ' name2 char(39)] ;
      |         str = sprintf('%s\ntext(.5,.5,%s,%s)',str1,name,str2) ;
      |         set_param(blk,'MaskDisplay',str) ;
      |     end
      |     clear value1 value2 expr name1 name2 name fcn1 fcn2 str1 str2 str
      | else
      |     cellarr(16:17) = {'off'} ;  val = get_param(blk,'MaskValues') ;
      |     for i=1:length(ind)
      |         a = findstr(val{ind(i)},'on') ;
      |         b(i) = isempty(a) ;
      |     end
      |     if isempty(find(b==0)) ;
      |         cellarr(ind) = {'on'} ;
      |     end
      | end
      | set_param(blk,'MaskVisibilities',cellarr) ;
      | clear blk value cellarr ind a b val i
      mask TypeOptions fromforce: Newtons | Dyne | Kilogram-Force | Ton-Force | Pound-Force
      mask Callback fromforce:
      | blk = gcb ;
      | value1 = get_param(blk,'fromforce') ;
      | value2 = get_param(blk,'toforce') ;
      | if strcmp(get_param(blk,'force'),'on') ;
      |     switch value1
      |         case 'Newtons'
      |             name1 = 'N' ;
      |             fcn1  = 'u(1)' ;
      |         case 'Dyne'
      |             name1 = 'dyne' ;
      |             fcn1  = 'u(1)*(1e-5)' ;
      |         case 'Kilogram-Force'
      |             name1 = 'kgf' ;
      |             fcn1  = 'u(1)*9.80665' ;
      |         case 'Ton-Force'
      |             name1 = 'tonf' ;
      |             fcn1  = 'u(1)*8896.44323052' ;
      |         case 'Pound-Force'
      |             name1 = 'lbf' ;
      |             fcn1  = 'u(1)*4.448221615' ;
      |     end
      |     switch value2
      |         case 'Newtons'
      |             name2 = 'N' ;
      |             fcn2  = '' ;
      |         case 'Dyne'
      |             name2 = 'dyne' ;
      |             fcn2  = '/(1e-5)' ;
      |         case 'Kilogram-Force'
      |             name2 = 'kgf' ;
      |             fcn2  = '/9.80665' ;
      |         case 'Ton-Force'
      |             name2 = 'tonf' ;
      |             fcn2  = '/8896.44323052' ;
      |         case 'Pound-Force'
      |             name2 = 'lbf' ;
      |             fcn2  = '/4.448221615' ;
      |     end
      |     expr = [fcn1 fcn2] ;
      |     %set_param(blk,'func',func) ;
      |     set_param([blk '/conv_fcn'],'expr',expr) ;
      |     str1 = ['% this block of text is updated via dialog callbacks'];
      |     str2 = [char(39) 'horizontalAlignment' char(39) ',' char(39) 'center' char(39) ',' char(39) 'texmode' char(39) ',' char(39) 'on' char(39)] ;
      |     name = [char(39) name1 ' to ' name2 char(39)] ;
      |     str = sprintf('%s\ntext(.5,.5,%s,%s)',str1,name,str2) ;
      |     set_param(blk,'MaskDisplay',str) ;
      | end
      |     clear blk value1 value2 expr name1 name2 name fcn1 fcn2 str1 str2 str
      mask TypeOptions toforce: Newtons | Dyne | Kilogram-Force | Ton-Force | Pound-Force
      mask Callback toforce:
      | blk = gcb ;
      | value1 = get_param(blk,'fromforce') ;
      | value2 = get_param(blk,'toforce') ;
      | if strcmp(get_param(blk,'force'),'on') ;
      |     switch value1
      |         case 'Newtons'
      |             name1 = 'N' ;
      |             fcn1  = 'u(1)' ;
      |         case 'Dyne'
      |             name1 = 'dyne' ;
      |             fcn1  = 'u(1)*(1e-5)' ;
      |         case 'Kilogram-Force'
      |             name1 = 'kgf' ;
      |             fcn1  = 'u(1)*9.80665' ;
      |         case 'Ton-Force'
      |             name1 = 'tonf' ;
      |             fcn1  = 'u(1)*8896.44323052' ;
      |         case 'Pound-Force'
      |             name1 = 'lbf' ;
      |             fcn1  = 'u(1)*4.448221615' ;
      |     end
      |     switch value2
      |         case 'Newtons'
      |             name2 = 'N' ;
      |             fcn2  = '' ;
      |         case 'Dyne'
      |             name2 = 'dyne' ;
      |             fcn2  = '/(1e-5)' ;
      |         case 'Kilogram-Force'
      |             name2 = 'kgf' ;
      |             fcn2  = '/9.80665' ;
      |         case 'Ton-Force'
      |             name2 = 'tonf' ;
      |             fcn2  = '/8896.44323052' ;
      |         case 'Pound-Force'
      |             name2 = 'lbf' ;
      |             fcn2  = '/4.448221615' ;
      |     end
      |     expr = [fcn1 fcn2] ;
      |     %set_param(blk,'func',func) ;
      |     set_param([blk '/conv_fcn'],'expr',expr) ;
      |     str1 = ['% this block of text is updated via dialog callbacks'];
      |     str2 = [char(39) 'horizontalAlignment' char(39) ',' char(39) 'center' char(39) ',' char(39) 'texmode' char(39) ',' char(39) 'on' char(39)] ;
      |     name = [char(39) name1 ' to ' name2 char(39)] ;
      |     str = sprintf('%s\ntext(.5,.5,%s,%s)',str1,name,str2) ;
      |     set_param(blk,'MaskDisplay',str) ;
      | end
      |     clear blk value1 value2 expr name1 name2 name fcn1 fcn2 str1 str2 str
      mask Callback temp:
      | blk = gcb ;
      | value = get_param(blk,'temp') ;
      | cellarr = get_param(blk,'MaskVisibilities') ;
      | ind = [1 4 9 12 15 18 21 24 27 30 33 38 43] ;
      | if strcmp(value,'on')
      |     cellarr(ind) = {'off'} ; cellarr(18:20) = {'on'} ;
      |     value1 = get_param(blk,'fromtemp') ;
      |     value2 = get_param(blk,'totemp') ;
      | 
      |     switch value1
      |         case 'Celcius'
      |             name1 = '{\circC}' ;
      |             fcn1  = '(u(1)+273.15)' ;
      |         case 'Kelvin'
      |             name1 = '{\circK}' ;
      |             fcn1  = 'u(1)' ;
      |         case 'Fahrenheit'
      |             name1 = '{\circF}' ;
      |             fcn1  = '(u(1)+459.67)/1.8' ;
      |         case 'Rankine'
      |             name1 = '{\circR}' ;
      |             fcn1  = 'u(1)/1.8' ;
      |     end
      |     switch value2
      |         case 'Celcius'
      |             name2 = '{\circC}' ;
      |             fcn2  = '-273.15'  ;
      |         case 'Kelvin'
      |             name2 = '{\circK}' ;
      |             fcn2  = '' ;
      |         case 'Fahrenheit'
      |             name2 = '{\circF}' ;
      |             fcn2  = '*1.8-459.67' ;
      |         case 'Rankine'
      |             name2 = '{\circR}' ;
      |             fcn2  = '*1.8' ;
      |     end
      |     expr = [fcn1 fcn2] ;
      |     %set_param(blk,'func',func) ;
      |     set_param([blk '/conv_fcn'],'expr',expr) ;
      |     str1 = ['% this block of text is updated via dialog callbacks'];
      |     str2 = [char(39) 'horizontalAlignment' char(39) ',' char(39) 'center' char(39) ',' char(39) 'texmode' char(39) ',' char(39) 'on' char(39)] ;
      |     name = [char(39) name1 ' to ' name2 char(39)] ;
      |     str = sprintf('%s\ntext(.5,.5,%s,%s)',str1,name,str2) ;
      |     set_param(blk,'MaskDisplay',str) ;
      |     clear value1 value2 expr name1 name2 name fcn1 fcn2 str1 str2 str
      | else
      |     cellarr(19:20) = {'off'} ; val = get_param(blk,'MaskValues') ;
      |     for i=1:length(ind)
      |         a = findstr(val{ind(i)},'on') ;
      |         b(i) = isempty(a) ;
      |     end
      |     if isempty(find(b==0)) ;
      |         cellarr(ind) = {'on'} ;
      |     end
      | end
      | set_param(blk,'MaskVisibilities',cellarr) ;
      | clear blk value cellarr ind a b val i
      mask TypeOptions fromtemp: Celcius | Kelvin | Fahrenheit | Rankine
      mask Callback fromtemp:
      | blk = gcb ;
      | value1 = get_param(blk,'fromtemp') ;
      | value2 = get_param(blk,'totemp') ;
      | if strcmp(get_param(blk,'temp'),'on') ;
      |     switch value1
      |         case 'Celcius'
      |             name1 = '{\circC}' ;
      |             fcn1  = '(u(1)+273.15)' ;
      |         case 'Kelvin'
      |             name1 = '{\circK}' ;
      |             fcn1  = 'u(1)' ;
      |         case 'Fahrenheit'
      |             name1 = '{\circF}' ;
      |             fcn1  = '(u(1)+459.67)/1.8' ;
      |         case 'Rankine'
      |             name1 = '{\circR}' ;
      |             fcn1  = 'u(1)/1.8' ;
      |     end
      |     switch value2
      |         case 'Celcius'
      |             name2 = '{\circC}' ;
      |             fcn2  = '-273.15'  ;
      |         case 'Kelvin'
      |             name2 = '{\circK}' ;
      |             fcn2  = '' ;
      |         case 'Fahrenheit'
      |             name2 = '{\circF}' ;
      |             fcn2  = '*1.8-459.67' ;
      |         case 'Rankine'
      |             name2 = '{\circR}' ;
      |             fcn2  = '*1.8' ;
      |     end
      |     expr = [fcn1 fcn2] ;
      |     %set_param(blk,'func',func) ;
      |     set_param([blk '/conv_fcn'],'expr',expr) ;
      |     str1 = ['% this block of text is updated via dialog callbacks'];
      |     str2 = [char(39) 'horizontalAlignment' char(39) ',' char(39) 'center' char(39) ',' char(39) 'texmode' char(39) ',' char(39) 'on' char(39)] ;
      |     name = [char(39) name1 ' to ' name2 char(39)] ;
      |     str = sprintf('%s\ntext(.5,.5,%s,%s)',str1,name,str2) ;
      |     set_param(blk,'MaskDisplay',str) ;
      | end
      |     clear blk value1 value2 expr name1 name2 name fcn1 fcn2 str1 str2 str
      mask TypeOptions totemp: Celcius | Kelvin | Fahrenheit | Rankine
      mask Callback totemp:
      | blk = gcb ;
      | value1 = get_param(blk,'fromtemp') ;
      | value2 = get_param(blk,'totemp') ;
      | if strcmp(get_param(blk,'temp'),'on') ;
      |     switch value1
      |         case 'Celcius'
      |             name1 = '{\circC}' ;
      |             fcn1  = '(u(1)+273.15)' ;
      |         case 'Kelvin'
      |             name1 = '{\circK}' ;
      |             fcn1  = 'u(1)' ;
      |         case 'Fahrenheit'
      |             name1 = '{\circF}' ;
      |             fcn1  = '(u(1)+459.67)/1.8' ;
      |         case 'Rankine'
      |             name1 = '{\circR}' ;
      |             fcn1  = 'u(1)/1.8' ;
      |     end
      |     switch value2
      |         case 'Celcius'
      |             name2 = '{\circC}' ;
      |             fcn2  = '-273.15'  ;
      |         case 'Kelvin'
      |             name2 = '{\circK}' ;
      |             fcn2  = '' ;
      |         case 'Fahrenheit'
      |             name2 = '{\circF}' ;
      |             fcn2  = '*1.8-459.67' ;
      |         case 'Rankine'
      |             name2 = '{\circR}' ;
      |             fcn2  = '*1.8' ;
      |     end
      |     expr = [fcn1 fcn2] ;
      |     %set_param(blk,'func',func) ;
      |     set_param([blk '/conv_fcn'],'expr',expr) ;
      |     str1 = ['% this block of text is updated via dialog callbacks'];
      |     str2 = [char(39) 'horizontalAlignment' char(39) ',' char(39) 'center' char(39) ',' char(39) 'texmode' char(39) ',' char(39) 'on' char(39)] ;
      |     name = [char(39) name1 ' to ' name2 char(39)] ;
      |     str = sprintf('%s\ntext(.5,.5,%s,%s)',str1,name,str2) ;
      |     set_param(blk,'MaskDisplay',str) ;
      | end
      |     clear blk value1 value2 expr name1 name2 name fcn1 fcn2 str1 str2 str
      mask Callback pres:
      | blk = gcb ;
      | value = get_param(blk,'pres') ;
      | cellarr = get_param(blk,'MaskVisibilities') ;
      | ind = [1 4 9 12 15 18 21 24 27 30 33 38 43] ;
      | if strcmp(value,'on') ;
      |     cellarr(ind) = {'off'} ; cellarr(21:23) = {'on'} ;
      |     value1 = get_param(blk,'frompres') ;
      |     value2 = get_param(blk,'topres') ;
      |     if strcmp(get_param(blk,'pres'),'on') ;
      |         switch value1
      |             case 'psia'
      |                 name1 = 'psia' ;
      |                 fcn1  = 'u(1)' ;
      |             case 'Pa'
      |                 name1 = 'Pa' ;
      |                 fcn1  = 'u(1)*(1.450377e-4)' ;
      |             case 'kPa'
      |                 name1 = 'kPa' ;
      |                 fcn1  = 'u(1)*(1.450377e-1)' ;
      |             case 'atm (0 C)'
      |                 name1 = 'atm' ;
      |                 fcn1  = 'u(1)*14.69595' ;
      |             case 'bar'
      |                 name1 = 'bar' ;
      |                 fcn1  = 'u(1)*14.503773773' ;
      |             case 'in Hg'
      |                 name1 = 'in Hg' ;
      |                 fcn1  = 'u(1)*.491154' ;
      |             case 'mm Hg'
      |                 name1 = 'mm Hg' ;
      |                 fcn1  = 'u(1)*.019336775' ;
      |             case 'in H20'
      |                 name1 = 'in H20' ;
      |                 fcn1  = 'u(1)*.036127292' ;
      |         end
      |         switch value2
      |             case 'psia'
      |                 name2 = 'psia' ;
      |                 fcn2  = '' ;
      |             case 'Pa'
      |                 name2 = 'Pa' ;
      |                 fcn2  = '/(1.450377e-4)' ;
      |             case 'kPa'
      |                 name2 = 'kPa' ;
      |                 fcn2  = '/(1.450377e-1)' ;
      |             case 'atm (0 C)'
      |                 name2 = 'atm' ;
      |                 fcn2  = '/14.69595' ;
      |             case 'bar'
      |                 name2 = 'bar' ;
      |                 fcn2  = '/14.503773773' ;
      |             case 'in Hg'
      |                 name2 = 'in Hg' ;
      |                 fcn2  = '/.491154' ;
      |             case 'mm Hg'
      |                 name2 = 'mm Hg' ;
      |                 fcn2  = '/.019336775' ;
      |             case 'in H20'
      |                 name2 = 'in H20' ;
      |                 fcn2  = '/.036127292' ;
      |         end
      |         expr = [fcn1 fcn2] ;
      |         %set_param(blk,'func',func) ;
      |         set_param([blk '/conv_fcn'],'expr',expr) ;
      |         str1 = ['% this block of text is updated via dialog callbacks'];
      |         str2 = [char(39) 'horizontalAlignment' char(39) ',' char(39) 'center' char(39) ',' char(39) 'texmode' char(39) ',' char(39) 'on' char(39)] ;
      |         name = [char(39) name1 ' to ' name2 char(39)] ;
      |         str = sprintf('%s\ntext(.5,.5,%s,%s)',str1,name,str2) ;
      |         set_param(blk,'MaskDisplay',str) ;
      |     end
      |     clear value1 value2 expr name1 name2 name fcn1 fcn2 str1 str2 str
      | else
      |     cellarr(22:23) = {'off'} ; val = get_param(blk,'MaskValues') ;
      |     for i=1:length(ind)
      |         a = findstr(val{ind(i)},'on') ;
      |         b(i) = isempty(a) ;
      |     end
      |     if isempty(find(b==0)) ;
      |         cellarr(ind) = {'on'} ;
      |     end
      | end
      | set_param(blk,'MaskVisibilities',cellarr) ;
      | clear blk value cellarr ind a b val i
      mask TypeOptions frompres: psia | Pa | kPa | atm (0 C) | bar | in Hg | mm Hg | in H20
      mask Callback frompres:
      | blk = gcb ;
      | value1 = get_param(blk,'frompres') ;
      | value2 = get_param(blk,'topres') ;
      | if strcmp(get_param(blk,'pres'),'on') ;
      |     switch value1
      |         case 'psia'
      |             name1 = 'psia' ;
      |             fcn1  = 'u(1)' ;
      |         case 'Pa'
      |             name1 = 'Pa' ;
      |             fcn1  = 'u(1)*(1.450377e-4)' ;
      |         case 'kPa'
      |             name1 = 'kPa' ;
      |             fcn1  = 'u(1)*(1.450377e-1)' ;
      |         case 'atm (0 C)'
      |             name1 = 'atm' ;
      |             fcn1  = 'u(1)*14.69595' ;
      |         case 'bar'
      |             name1 = 'bar' ;
      |             fcn1  = 'u(1)*14.503773773' ;
      |         case 'in Hg'
      |             name1 = 'in Hg' ;
      |             fcn1  = 'u(1)*.491154' ;
      |         case 'mm Hg'
      |             name1 = 'mm Hg' ;
      |             fcn1  = 'u(1)*.019336775' ;
      |         case 'in H20'
      |             name1 = 'in H20' ;
      |             fcn1  = 'u(1)*.036127292' ;
      |     end
      |     switch value2
      |         case 'psia'
      |             name2 = 'psia' ;
      |             fcn2  = '' ;
      |         case 'Pa'
      |             name2 = 'Pa' ;
      |             fcn2  = '/(1.450377e-4)' ;
      |         case 'kPa'
      |             name2 = 'kPa' ;
      |             fcn2  = '/(1.450377e-1)' ;
      |         case 'atm (0 C)'
      |             name2 = 'atm' ;
      |             fcn2  = '/14.69595' ;
      |         case 'bar'
      |             name2 = 'bar' ;
      |             fcn2  = '/14.503773773' ;
      |         case 'in Hg'
      |             name2 = 'in Hg' ;
      |             fcn2  = '/.491154' ;
      |         case 'mm Hg'
      |             name2 = 'mm Hg' ;
      |             fcn2  = '/.019336775' ;
      |         case 'in H20'
      |             name2 = 'in H20' ;
      |             fcn2  = '/.036127292' ;
      |     end
      |     expr = [fcn1 fcn2] ;
      |     %set_param(blk,'func',func) ;
      |     set_param([blk '/conv_fcn'],'expr',expr) ;
      |     str1 = ['% this block of text is updated via dialog callbacks'];
      |     str2 = [char(39) 'horizontalAlignment' char(39) ',' char(39) 'center' char(39) ',' char(39) 'texmode' char(39) ',' char(39) 'on' char(39)] ;
      |     name = [char(39) name1 ' to ' name2 char(39)] ;
      |     str = sprintf('%s\ntext(.5,.5,%s,%s)',str1,name,str2) ;
      |     set_param(blk,'MaskDisplay',str) ;
      | end
      |     clear blk value1 value2 expr name1 name2 name fcn1 fcn2 str1 str2 str
      mask TypeOptions topres: psia | Pa | kPa | atm (0 C) | bar | in Hg | mm Hg | in H20
      mask Callback topres:
      | blk = gcb ;
      | value1 = get_param(blk,'frompres') ;
      | value2 = get_param(blk,'topres') ;
      | if strcmp(get_param(blk,'pres'),'on') ;
      |     switch value1
      |         case 'psia'
      |             name1 = 'psia' ;
      |             fcn1  = 'u(1)' ;
      |         case 'Pa'
      |             name1 = 'Pa' ;
      |             fcn1  = 'u(1)*(1.450377e-4)' ;
      |         case 'kPa'
      |             name1 = 'kPa' ;
      |             fcn1  = 'u(1)*(1.450377e-1)' ;
      |         case 'atm (0 C)'
      |             name1 = 'atm' ;
      |             fcn1  = 'u(1)*14.69595' ;
      |         case 'bar'
      |             name1 = 'bar' ;
      |             fcn1  = 'u(1)*14.503773773' ;
      |         case 'in Hg'
      |             name1 = 'in Hg' ;
      |             fcn1  = 'u(1)*.491154' ;
      |         case 'mm Hg'
      |             name1 = 'mm Hg' ;
      |             fcn1  = 'u(1)*.019336775' ;
      |         case 'in H20'
      |             name1 = 'in H20' ;
      |             fcn1  = 'u(1)*.036127292' ;
      |     end
      |     switch value2
      |         case 'psia'
      |             name2 = 'psia' ;
      |             fcn2  = '' ;
      |         case 'Pa'
      |             name2 = 'Pa' ;
      |             fcn2  = '/(1.450377e-4)' ;
      |         case 'kPa'
      |             name2 = 'kPa' ;
      |             fcn2  = '/(1.450377e-1)' ;
      |         case 'atm (0 C)'
      |             name2 = 'atm' ;
      |             fcn2  = '/14.69595' ;
      |         case 'bar'
      |             name2 = 'bar' ;
      |             fcn2  = '/14.503773773' ;
      |         case 'in Hg'
      |             name2 = 'in Hg' ;
      |             fcn2  = '/.491154' ;
      |         case 'mm Hg'
      |             name2 = 'mm Hg' ;
      |             fcn2  = '/.019336775' ;
      |         case 'in H20'
      |             name2 = 'in H20' ;
      |             fcn2  = '/.036127292' ;
      |     end
      |     expr = [fcn1 fcn2] ;
      |     %set_param(blk,'func',func) ;
      |     set_param([blk '/conv_fcn'],'expr',expr) ;
      |     str1 = ['% this block of text is updated via dialog callbacks'];
      |     str2 = [char(39) 'horizontalAlignment' char(39) ',' char(39) 'center' char(39) ',' char(39) 'texmode' char(39) ',' char(39) 'on' char(39)] ;
      |     name = [char(39) name1 ' to ' name2 char(39)] ;
      |     str = sprintf('%s\ntext(.5,.5,%s,%s)',str1,name,str2) ;
      |     set_param(blk,'MaskDisplay',str) ;
      | end
      |     clear blk value1 value2 expr name1 name2 name fcn1 fcn2 str1 str2 str
      mask Callback length:
      | blk = gcb ;
      | value = get_param(blk,'length') ;
      | cellarr = get_param(blk,'MaskVisibilities') ;
      | ind = [1 4 9 12 15 18 21 24 27 30 33 38 43] ;
      | if strcmp(value,'on')
      |     cellarr(ind) = {'off'} ; cellarr(24:26) = {'on'} ;
      |     value1 = get_param(blk,'fromlength') ;
      |     value2 = get_param(blk,'tolength') ;
      |     if strcmp(get_param(blk,'length'),'on') ;
      |         switch value1
      |             case 'Millimeters'
      |                 name1 = 'mm' ;
      |                 fcn1  = 'u(1)*.001' ;
      |             case 'Centimeters'
      |                 name1 = 'cm' ;
      |                 fcn1  = 'u(1)*.01' ;
      |             case 'Meters'
      |                 name1 = 'm' ;
      |                 fcn1  = 'u(1)' ;
      |             case 'Kilometers'
      |                 name1 = 'km' ;
      |                 fcn1  = 'u(1)/1000' ;
      |             case 'Inches'
      |                 name1 = 'in' ;
      |                 fcn1  = 'u(1)*.0254' ;
      |             case 'Feet'
      |                 name1 = 'ft' ;
      |                 fcn1  = 'u(1)*.3048' ;
      |             case 'Yards'
      |                 name1 = 'yd' ;
      |                 fcn1  = 'u(1)*.9144' ;
      |             case 'Miles'
      |                 name1 = 'mi' ;
      |                 fcn1  = 'u(1)*1609.344' ;
      |             case 'Nautical Miles'
      |                 name1 = 'nmi' ;
      |                 fcn1  = 'u(1)*1852' ;
      |         end
      |         switch value2
      |             case 'Millimeters'
      |                 name2 = 'mm' ;
      |                 fcn2  = '/.001' ;
      |             case 'Centimeters'
      |                 name2 = 'cm' ;
      |                 fcn2 = '/.01' ;
      |             case 'Meters'
      |                 name2 = 'm' ;
      |                 fcn2  = '' ;
      |             case 'Kilometers'
      |                 name2 = 'km' ;
      |                 fcn2  = '/1000' ;
      |             case 'Inches'
      |                 name2 = 'in' ;
      |                 fcn2  = '/.0254' ;
      |             case 'Feet'
      |                 name2 = 'ft' ;
      |                 fcn2  = '/.3048' ;
      |             case 'Yards'
      |                 name2 = 'yd' ;
      |                 fcn2  = '/.9144' ;
      |             case 'Miles'
      |                 name2 = 'mi' ;
      |                 fcn2  = '/1609.344' ;
      |             case 'Nautical Miles'
      |                 name2 = 'nmi' ;
      |                 fcn2  = '/1852' ;
      |         end
      |         expr = [fcn1 fcn2] ;
      |         %set_param(blk,'func',func) ;
      |         set_param([blk '/conv_fcn'],'expr',expr) ;
      |         str1 = ['% this block of text is updated via dialog callbacks'];
      |         str2 = [char(39) 'horizontalAlignment' char(39) ',' char(39) 'center' char(39) ',' char(39) 'texmode' char(39) ',' char(39) 'on' char(39)] ;
      |         name = [char(39) name1 ' to ' name2 char(39)] ;
      |         str = sprintf('%s\ntext(.5,.5,%s,%s)',str1,name,str2) ;
      |         set_param(blk,'MaskDisplay',str) ;
      |     end
      |     clear value1 value2 expr name1 name2 name fcn1 fcn2 str1 str2 str
      | else
      |     cellarr(25:26) = {'off'} ; val = get_param(blk,'MaskValues') ;
      |     for i=1:length(ind)
      |         a = findstr(val{ind(i)},'on') ;
      |         b(i) = isempty(a) ;
      |     end
      |     if isempty(find(b==0)) ;
      |         cellarr(ind) = {'on'} ;
      |     end
      | end
      | set_param(blk,'MaskVisibilities',cellarr) ;
      | clear blk value cellarr ind a b val i
      mask TypeOptions fromlength: Millimeters | Centimeters | Meters | Kilometers | Inches | Feet | Yards | Miles | Nautical Miles
      mask Callback fromlength:
      | blk = gcb ;
      | value1 = get_param(blk,'fromlength') ;
      | value2 = get_param(blk,'tolength') ;
      | if strcmp(get_param(blk,'length'),'on') ;
      |     switch value1
      |         case 'Millimeters'
      |             name1 = 'mm' ;
      |             fcn1  = 'u(1)*.001' ;
      |         case 'Centimeters'
      |             name1 = 'cm' ;
      |             fcn1  = 'u(1)*.01' ;
      |         case 'Meters'
      |             name1 = 'm' ;
      |             fcn1  = 'u(1)' ;
      |         case 'Kilometers'
      |             name1 = 'km' ;
      |             fcn1  = 'u(1)/1000' ;
      |         case 'Inches'
      |             name1 = 'in' ;
      |             fcn1  = 'u(1)*.0254' ;
      |         case 'Feet'
      |             name1 = 'ft' ;
      |             fcn1  = 'u(1)*.3048' ;
      |         case 'Yards'
      |             name1 = 'yd' ;
      |             fcn1  = 'u(1)*.9144' ;
      |         case 'Miles'
      |             name1 = 'mi' ;
      |             fcn1  = 'u(1)*1609.344' ;
      |         case 'Nautical Miles'
      |             name1 = 'nmi' ;
      |             fcn1  = 'u(1)*1852' ;
      |     end
      |     switch value2
      |         case 'Millimeters'
      |             name2 = 'mm' ;
      |             fcn2  = '/.001' ;
      |         case 'Centimeters'
      |             name2 = 'cm' ;
      |             fcn2 = '/.01' ;
      |         case 'Meters'
      |             name2 = 'm' ;
      |             fcn2  = '' ;
      |         case 'Kilometers'
      |             name2 = 'km' ;
      |             fcn2  = '/1000' ;
      |         case 'Inches'
      |             name2 = 'in' ;
      |             fcn2  = '/.0254' ;
      |         case 'Feet'
      |             name2 = 'ft' ;
      |             fcn2  = '/.3048' ;
      |         case 'Yards'
      |             name2 = 'yd' ;
      |             fcn2  = '/.9144' ;
      |         case 'Miles'
      |             name2 = 'mi' ;
      |             fcn2  = '/1609.344' ;
      |         case 'Nautical Miles'
      |             name2 = 'nmi' ;
      |             fcn2  = '/1852' ;
      |     end
      |     expr = [fcn1 fcn2] ;
      |     %set_param(blk,'func',func) ;
      |     set_param([blk '/conv_fcn'],'expr',expr) ;
      |     str1 = ['% this block of text is updated via dialog callbacks'];
      |     str2 = [char(39) 'horizontalAlignment' char(39) ',' char(39) 'center' char(39) ',' char(39) 'texmode' char(39) ',' char(39) 'on' char(39)] ;
      |     name = [char(39) name1 ' to ' name2 char(39)] ;
      |     str = sprintf('%s\ntext(.5,.5,%s,%s)',str1,name,str2) ;
      |     set_param(blk,'MaskDisplay',str) ;
      | end
      | clear blk value1 value2 expr name1 name2 name fcn1 fcn2 str1 str2 str
      mask TypeOptions tolength: Millimeters | Centimeters | Meters | Kilometers | Inches | Feet | Yards | Miles | Nautical Miles
      mask Callback tolength:
      | blk = gcb ;
      | value1 = get_param(blk,'fromlength') ;
      | value2 = get_param(blk,'tolength') ;
      | if strcmp(get_param(blk,'length'),'on') ;
      |     switch value1
      |         case 'Millimeters'
      |             name1 = 'mm' ;
      |             fcn1  = 'u(1)*.001' ;
      |         case 'Centimeters'
      |             name1 = 'cm' ;
      |             fcn1  = 'u(1)*.01' ;
      |         case 'Meters'
      |             name1 = 'm' ;
      |             fcn1  = 'u(1)' ;
      |         case 'Kilometers'
      |             name1 = 'km' ;
      |             fcn1  = 'u(1)/1000' ;
      |         case 'Inches'
      |             name1 = 'in' ;
      |             fcn1  = 'u(1)*.0254' ;
      |         case 'Feet'
      |             name1 = 'ft' ;
      |             fcn1  = 'u(1)*.3048' ;
      |         case 'Yards'
      |             name1 = 'yd' ;
      |             fcn1  = 'u(1)*.9144' ;
      |         case 'Miles'
      |             name1 = 'mi' ;
      |             fcn1  = 'u(1)*1609.344' ;
      |         case 'Nautical Miles'
      |             name1 = 'nmi' ;
      |             fcn1  = 'u(1)*1852' ;
      |     end
      |     switch value2
      |         case 'Millimeters'
      |             name2 = 'mm' ;
      |             fcn2  = '/.001' ;
      |         case 'Centimeters'
      |             name2 = 'cm' ;
      |             fcn2 = '/.01' ;
      |         case 'Meters'
      |             name2 = 'm' ;
      |             fcn2  = '' ;
      |         case 'Kilometers'
      |             name2 = 'km' ;
      |             fcn2  = '/1000' ;
      |         case 'Inches'
      |             name2 = 'in' ;
      |             fcn2  = '/.0254' ;
      |         case 'Feet'
      |             name2 = 'ft' ;
      |             fcn2  = '/.3048' ;
      |         case 'Yards'
      |             name2 = 'yd' ;
      |             fcn2  = '/.9144' ;
      |         case 'Miles'
      |             name2 = 'mi' ;
      |             fcn2  = '/1609.344' ;
      |         case 'Nautical Miles'
      |             name2 = 'nmi' ;
      |             fcn2  = '/1852' ;
      |     end
      |     expr = [fcn1 fcn2] ;
      |     %set_param(blk,'func',func) ;
      |     set_param([blk '/conv_fcn'],'expr',expr) ;
      |     str1 = ['% this block of text is updated via dialog callbacks'];
      |     str2 = [char(39) 'horizontalAlignment' char(39) ',' char(39) 'center' char(39) ',' char(39) 'texmode' char(39) ',' char(39) 'on' char(39)] ;
      |     name = [char(39) name1 ' to ' name2 char(39)] ;
      |     str = sprintf('%s\ntext(.5,.5,%s,%s)',str1,name,str2) ;
      |     set_param(blk,'MaskDisplay',str) ;
      | end
      | clear blk value1 value2 expr name1 name2 name fcn1 fcn2 str1 str2 str
      mask Callback area:
      | blk = gcb ;
      | value = get_param(blk,'area') ;
      | cellarr = get_param(blk,'MaskVisibilities');
      | ind = [1 4 9 12 15 18 21 24 27 30 33 38 43] ;
      | if strcmp(value,'on')
      |     cellarr(ind) = {'off'} ; cellarr(27:29) = {'on'} ;
      |     value1 = get_param(blk,'fromarea') ;
      |     value2 = get_param(blk,'toarea') ;
      |     if strcmp(get_param(blk,'area'),'on') ;
      |         switch value1
      |             case 'Square Centimeters'
      |                 name1 = 'cm^2' ;
      |                 fcn1  = 'u(1)*(1e-4)' ;
      |             case 'Square Meters'
      |                 name1 = 'm^2' ;
      |                 fcn1  = 'u(1)' ;
      |             case 'Square Kilometers'
      |                 name1 = 'km^2' ;
      |                 fcn1  = 'u(1)*(1e6)' ;
      |             case 'Square Inches'
      |                 name1 = 'in^2' ;
      |                 fcn1  = 'u(1)*6.4516e-4' ;
      |             case 'Square Feet'
      |                 name1 = 'ft^2' ;
      |                 fcn1  = 'u(1)*.09290304' ;
      |             case 'Square Yards'
      |                 name1 = 'yd^2' ;
      |                 fcn1  = 'u(1)*.83612736' ;
      |             case 'Acres'
      |                 name1 = 'acre' ;
      |                 fcn1  = 'u(1)*4046.8564224' ;
      |             case 'Square Miles'
      |                 name1 = 'mi^2' ;
      |                 fcn1  = 'u(1)*(2.589988e6)' ;
      |         end
      |         switch value2
      |             case 'Square Centimeters'
      |                 name2 = 'cm^2' ;
      |                 fcn2  = '/(1e-4)' ;
      |             case 'Square Meters'
      |                 name2 = 'm^2' ;
      |                 fcn2  = '' ;
      |             case 'Square Kilometers'
      |                 name2 = 'km^2' ;
      |                 fcn2  = '/(1e6)' ;
      |             case 'Square Inches'
      |                 name2 = 'in^2' ;
      |                 fcn2  = '/6.4516e-4' ;
      |             case 'Square Feet'
      |                 name2 = 'ft^2' ;
      |                 fcn2  = '/.09290304' ;
      |             case 'Square Yards'
      |                 name2 = 'yd^2' ;
      |                 fcn2  = '/.83612736' ;
      |             case 'Acres'
      |                 name2 = 'acre' ;
      |                 fcn2  = '/4046.8564224' ;
      |             case 'Square Miles'
      |                 name2 = 'mi^2' ;
      |                 fcn2  = '/(2.589988e6)' ;
      |         end
      |         expr = [fcn1 fcn2] ;
      |         %set_param(blk,'func',func) ;
      |         set_param([blk '/conv_fcn'],'expr',expr) ;
      |         str1 = ['% this block of text is updated via dialog callbacks'];
      |         str2 = [char(39) 'horizontalAlignment' char(39) ',' char(39) 'center' char(39) ',' char(39) 'texmode' char(39) ',' char(39) 'on' char(39)] ;
      |         name = [char(39) name1 ' to ' name2 char(39)] ;
      |         str = sprintf('%s\ntext(.5,.5,%s,%s)',str1,name,str2) ;
      |         set_param(blk,'MaskDisplay',str) ;
      |     end
      |     clear value1 value2 expr name1 name2 name fcn1 fcn2 str1 str2 str
      | else
      |     cellarr(28:29) = {'off'} ; val = get_param(blk,'MaskValues') ;
      |     for i=1:length(ind)
      |         a = findstr(val{ind(i)},'on') ;
      |         b(i) = isempty(a) ;
      |     end
      |     if isempty(find(b==0)) ;
      |         cellarr(ind) = {'on'} ;
      |     end
      | end
      | set_param(blk,'MaskVisibilities',cellarr) ;
      | clear blk value cellarr ind a b val i
      mask TypeOptions fromarea: Square Centimeters | Square Meters | Square Kilometers | Square Inches | Square Feet | Square Yards | Acres | Square Miles
      mask Callback fromarea:
      | blk = gcb ;
      | value1 = get_param(blk,'fromarea') ;
      | value2 = get_param(blk,'toarea') ;
      | if strcmp(get_param(blk,'area'),'on') ;
      |     switch value1
      |         case 'Square Centimeters'
      |             name1 = 'cm^2' ;
      |             fcn1  = 'u(1)*(1e-4)' ;
      |         case 'Square Meters'
      |             name1 = 'm^2' ;
      |             fcn1  = 'u(1)' ;
      |         case 'Square Kilometers'
      |             name1 = 'km^2' ;
      |             fcn1  = 'u(1)*(1e6)' ;
      |         case 'Square Inches'
      |             name1 = 'in^2' ;
      |             fcn1  = 'u(1)*6.4516e-4' ;
      |         case 'Square Feet'
      |             name1 = 'ft^2' ;
      |             fcn1  = 'u(1)*.09290304' ;
      |         case 'Square Yards'
      |             name1 = 'yd^2' ;
      |             fcn1  = 'u(1)*.83612736' ;
      |         case 'Acres'
      |             name1 = 'acre' ;
      |             fcn1  = 'u(1)*4046.8564224' ;
      |         case 'Square Miles'
      |             name1 = 'mi^2' ;
      |             fcn1  = 'u(1)*(2.589988e6)' ;
      |     end
      |     switch value2
      |         case 'Square Centimeters'
      |             name2 = 'cm^2' ;
      |             fcn2  = '/(1e-4)' ;
      |         case 'Square Meters'
      |             name2 = 'm^2' ;
      |             fcn2  = '' ;
      |         case 'Square Kilometers'
      |             name2 = 'km^2' ;
      |             fcn2  = '/(1e6)' ;
      |         case 'Square Inches'
      |             name2 = 'in^2' ;
      |             fcn2  = '/6.4516e-4' ;
      |         case 'Square Feet'
      |             name2 = 'ft^2' ;
      |             fcn2  = '/.09290304' ;
      |         case 'Square Yards'
      |             name2 = 'yd^2' ;
      |             fcn2  = '/.83612736' ;
      |         case 'Acres'
      |             name2 = 'acre' ;
      |             fcn2  = '/4046.8564224' ;
      |         case 'Square Miles'
      |             name2 = 'mi^2' ;
      |             fcn2  = '/(2.589988e6)' ;
      |     end
      |     expr = [fcn1 fcn2] ;
      |     %set_param(blk,'func',func) ;
      |     set_param([blk '/conv_fcn'],'expr',expr) ;
      |     str1 = ['% this block of text is updated via dialog callbacks'];
      |     str2 = [char(39) 'horizontalAlignment' char(39) ',' char(39) 'center' char(39) ',' char(39) 'texmode' char(39) ',' char(39) 'on' char(39)] ;
      |     name = [char(39) name1 ' to ' name2 char(39)] ;
      |     str = sprintf('%s\ntext(.5,.5,%s,%s)',str1,name,str2) ;
      |     set_param(blk,'MaskDisplay',str) ;
      | end
      |     clear blk value1 value2 expr name1 name2 name fcn1 fcn2 str1 str2 str
      mask TypeOptions toarea: Square Centimeters | Square Meters | Square Kilometers | Square Inches | Square Feet | Square Yards | Acres | Square Miles
      mask Callback toarea:
      | blk = gcb ;
      | value1 = get_param(blk,'fromarea') ;
      | value2 = get_param(blk,'toarea') ;
      | if strcmp(get_param(blk,'area'),'on') ;
      |     switch value1
      |         case 'Square Centimeters'
      |             name1 = 'cm^2' ;
      |             fcn1  = 'u(1)*(1e-4)' ;
      |         case 'Square Meters'
      |             name1 = 'm^2' ;
      |             fcn1  = 'u(1)' ;
      |         case 'Square Kilometers'
      |             name1 = 'km^2' ;
      |             fcn1  = 'u(1)*(1e6)' ;
      |         case 'Square Inches'
      |             name1 = 'in^2' ;
      |             fcn1  = 'u(1)*6.4516e-4' ;
      |         case 'Square Feet'
      |             name1 = 'ft^2' ;
      |             fcn1  = 'u(1)*.09290304' ;
      |         case 'Square Yards'
      |             name1 = 'yd^2' ;
      |             fcn1  = 'u(1)*.83612736' ;
      |         case 'Acres'
      |             name1 = 'acre' ;
      |             fcn1  = 'u(1)*4046.8564224' ;
      |         case 'Square Miles'
      |             name1 = 'mi^2' ;
      |             fcn1  = 'u(1)*(2.589988e6)' ;
      |     end
      |     switch value2
      |         case 'Square Centimeters'
      |             name2 = 'cm^2' ;
      |             fcn2  = '/(1e-4)' ;
      |         case 'Square Meters'
      |             name2 = 'm^2' ;
      |             fcn2  = '' ;
      |         case 'Square Kilometers'
      |             name2 = 'km^2' ;
      |             fcn2  = '/(1e6)' ;
      |         case 'Square Inches'
      |             name2 = 'in^2' ;
      |             fcn2  = '/6.4516e-4' ;
      |         case 'Square Feet'
      |             name2 = 'ft^2' ;
      |             fcn2  = '/.09290304' ;
      |         case 'Square Yards'
      |             name2 = 'yd^2' ;
      |             fcn2  = '/.83612736' ;
      |         case 'Acres'
      |             name2 = 'acre' ;
      |             fcn2  = '/4046.8564224' ;
      |         case 'Square Miles'
      |             name2 = 'mi^2' ;
      |             fcn2  = '/(2.589988e6)' ;
      |     end
      |     expr = [fcn1 fcn2] ;
      |     %set_param(blk,'func',func) ;
      |     set_param([blk '/conv_fcn'],'expr',expr) ;
      |     str1 = ['% this block of text is updated via dialog callbacks'];
      |     str2 = [char(39) 'horizontalAlignment' char(39) ',' char(39) 'center' char(39) ',' char(39) 'texmode' char(39) ',' char(39) 'on' char(39)] ;
      |     name = [char(39) name1 ' to ' name2 char(39)] ;
      |     str = sprintf('%s\ntext(.5,.5,%s,%s)',str1,name,str2) ;
      |     set_param(blk,'MaskDisplay',str) ;
      | end
      |     clear blk value1 value2 expr name1 name2 name fcn1 fcn2 str1 str2 str
      mask Callback vol:
      | blk = gcb ;
      | value = get_param(blk,'vol') ;
      | cellarr = get_param(blk,'MaskVisibilities') ;
      | ind = [1 4 9 12 15 18 21 24 27 30 33 38 43] ;
      | if strcmp(value,'on') ;
      |     cellarr(ind) = {'off'} ; cellarr(30:32) = {'on'} ;
      |     value1 = get_param(blk,'fromvol') ;
      |     value2 = get_param(blk,'tovol') ;
      |     if strcmp(get_param(blk,'vol'),'on') ;
      |         switch value1
      |             case 'Milliliters'
      |                 name1 = 'mL' ;
      |                 fcn1  = 'u(1)*(1e-6)' ;
      |             case 'Liters'
      |                 name1 = 'L' ;
      |                 fcn1  = 'u(1)*.001' ;
      |             case 'Cubic Centimeters'
      |                 name1 = 'cm^3' ;
      |                 fcn1  = 'u(1)*(1e-6)' ;
      |             case 'Cubic Meters'
      |                 name1 = 'm^3' ;
      |                 fcn1  = 'u(1)' ;
      |             case 'Ounces'
      |                 name1 = 'oz' ;
      |                 fcn1  = 'u(1)*(2.95735e-5)' ;
      |             case 'Gallons'
      |                 name1 = 'gal' ;
      |                 fcn1  = 'u(1)*.0037854' ;
      |             case 'Cubic Inches'
      |                 name1 = 'in^3' ;
      |                 fcn1  = 'u(1)*(1.6387e-5)' ;
      |             case 'Cubic Feet'
      |                 name1 = 'ft^3' ;
      |                 fcn1  = 'u(1)*.02831685' ;
      |         end
      |         switch value2
      |             case 'Milliliters'
      |                 name2 = 'mL' ;
      |                 fcn2  = '/(1e-6)' ;
      |             case 'Liters'
      |                 name2 = 'L' ;
      |                 fcn2  = '/.001' ;
      |             case 'Cubic Centimeters'
      |                 name2 = 'cm^3' ;
      |                 fcn2  = '/(1e-6)' ;
      |             case 'Cubic Meters'
      |                 name2 = 'm^3' ;
      |                 fcn2  = '' ;
      |             case 'Ounces'
      |                 name2 = 'oz' ;
      |                 fcn2  = '/(2.95735e-5)' ;
      |             case 'Gallons'
      |                 name2 = 'gal' ;
      |                 fcn2  = '/.0037854' ;
      |             case 'Cubic Inches'
      |                 name2 = 'in^3' ;
      |                 fcn2  = '/(1.6387e-5)' ;
      |             case 'Cubic Feet'
      |                 name2 = 'ft^3' ;
      |                 fcn2  = '/.02831685' ;
      |         end
      |         expr = [fcn1 fcn2] ;
      |         %set_param(blk,'func',func) ;
      |         set_param([blk '/conv_fcn'],'expr',expr) ;
      |         str1 = ['% this block of text is updated via dialog callbacks'];
      |         str2 = [char(39) 'horizontalAlignment' char(39) ',' char(39) 'center' char(39) ',' char(39) 'texmode' char(39) ',' char(39) 'on' char(39)] ;
      |         name = [char(39) name1 ' to ' name2 char(39)] ;
      |         str = sprintf('%s\ntext(.5,.5,%s,%s)',str1,name,str2) ;
      |         set_param(blk,'MaskDisplay',str) ;
      |     end
      |     clear  value1 value2 expr name1 name2 name fcn1 fcn2 str1 str2 str
      | else
      |     cellarr(31:32) = {'off'} ; val = get_param(blk,'MaskValues') ;
      |     for i=1:length(ind)
      |         a = findstr(val{ind(i)},'on') ;
      |         b(i) = isempty(a) ;
      |     end
      |     if isempty(find(b==0)) ;
      |         cellarr(ind) = {'on'} ;
      |     end
      | end
      | set_param(blk,'MaskVisibilities',cellarr) ;
      | clear blk value cellarr ind a b val i
      mask TypeOptions fromvol: Milliliters | Liters | Cubic Centimeters | Cubic Meters | Ounces | Gallons | Cubic Inches | Cubic Feet
      mask Callback fromvol:
      | blk = gcb ;
      | value1 = get_param(blk,'fromvol') ;
      | value2 = get_param(blk,'tovol') ;
      | if strcmp(get_param(blk,'vol'),'on') ;
      |     switch value1
      |         case 'Milliliters'
      |             name1 = 'mL' ;
      |             fcn1  = 'u(1)*(1e-6)' ;
      |         case 'Liters'
      |             name1 = 'L' ;
      |             fcn1  = 'u(1)*.001' ;
      |         case 'Cubic Centimeters'
      |             name1 = 'cm^3' ;
      |             fcn1  = 'u(1)*(1e-6)' ;
      |         case 'Cubic Meters'
      |             name1 = 'm^3' ;
      |             fcn1  = 'u(1)' ;
      |         case 'Ounces'
      |             name1 = 'oz' ;
      |             fcn1  = 'u(1)*(2.95735e-5)' ;
      |         case 'Gallons'
      |             name1 = 'gal' ;
      |             fcn1  = 'u(1)*.0037854' ;
      |         case 'Cubic Inches'
      |             name1 = 'in^3' ;
      |             fcn1  = 'u(1)*(1.6387e-5)' ;
      |         case 'Cubic Feet'
      |             name1 = 'ft^3' ;
      |             fcn1  = 'u(1)*.02831685' ;
      |     end
      |     switch value2
      |         case 'Milliliters'
      |             name2 = 'mL' ;
      |             fcn2  = '/(1e-6)' ;
      |         case 'Liters'
      |             name2 = 'L' ;
      |             fcn2  = '/.001' ;
      |         case 'Cubic Centimeters'
      |             name2 = 'cm^3' ;
      |             fcn2  = '/(1e-6)' ;
      |         case 'Cubic Meters'
      |             name2 = 'm^3' ;
      |             fcn2  = '' ;
      |         case 'Ounces'
      |             name2 = 'oz' ;
      |             fcn2  = '/(2.95735e-5)' ;
      |         case 'Gallons'
      |             name2 = 'gal' ;
      |             fcn2  = '/.0037854' ;
      |         case 'Cubic Inches'
      |             name2 = 'in^3' ;
      |             fcn2  = '/(1.6387e-5)' ;
      |         case 'Cubic Feet'
      |             name2 = 'ft^3' ;
      |             fcn2  = '/.02831685' ;
      |     end
      |     expr = [fcn1 fcn2] ;
      |     %set_param(blk,'func',func) ;
      |     set_param([blk '/conv_fcn'],'expr',expr) ;
      |     str1 = ['% this block of text is updated via dialog callbacks'];
      |     str2 = [char(39) 'horizontalAlignment' char(39) ',' char(39) 'center' char(39) ',' char(39) 'texmode' char(39) ',' char(39) 'on' char(39)] ;
      |     name = [char(39) name1 ' to ' name2 char(39)] ;
      |     str = sprintf('%s\ntext(.5,.5,%s,%s)',str1,name,str2) ;
      |     set_param(blk,'MaskDisplay',str) ;
      | end
      |     clear blk value1 value2 expr name1 name2 name fcn1 fcn2 str1 str2 str
      mask TypeOptions tovol: Milliliters | Liters | Cubic Centimeters | Cubic Meters | Ounces | Gallons | Cubic Inches | Cubic Feet
      mask Callback tovol:
      | blk = gcb ;
      | value1 = get_param(blk,'fromvol') ;
      | value2 = get_param(blk,'tovol') ;
      | if strcmp(get_param(blk,'vol'),'on') ;
      |     switch value1
      |         case 'Milliliters'
      |             name1 = 'mL' ;
      |             fcn1  = 'u(1)*(1e-6)' ;
      |         case 'Liters'
      |             name1 = 'L' ;
      |             fcn1  = 'u(1)*.001' ;
      |         case 'Cubic Centimeters'
      |             name1 = 'cm^3' ;
      |             fcn1  = 'u(1)*(1e-6)' ;
      |         case 'Cubic Meters'
      |             name1 = 'm^3' ;
      |             fcn1  = 'u(1)' ;
      |         case 'Ounces'
      |             name1 = 'oz' ;
      |             fcn1  = 'u(1)*(2.95735e-5)' ;
      |         case 'Gallons'
      |             name1 = 'gal' ;
      |             fcn1  = 'u(1)*.0037854' ;
      |         case 'Cubic Inches'
      |             name1 = 'in^3' ;
      |             fcn1  = 'u(1)*(1.6387e-5)' ;
      |         case 'Cubic Feet'
      |             name1 = 'ft^3' ;
      |             fcn1  = 'u(1)*.02831685' ;
      |     end
      |     switch value2
      |         case 'Milliliters'
      |             name2 = 'mL' ;
      |             fcn2  = '/(1e-6)' ;
      |         case 'Liters'
      |             name2 = 'L' ;
      |             fcn2  = '/.001' ;
      |         case 'Cubic Centimeters'
      |             name2 = 'cm^3' ;
      |             fcn2  = '/(1e-6)' ;
      |         case 'Cubic Meters'
      |             name2 = 'm^3' ;
      |             fcn2  = '' ;
      |         case 'Ounces'
      |             name2 = 'oz' ;
      |             fcn2  = '/(2.95735e-5)' ;
      |         case 'Gallons'
      |             name2 = 'gal' ;
      |             fcn2  = '/.0037854' ;
      |         case 'Cubic Inches'
      |             name2 = 'in^3' ;
      |             fcn2  = '/(1.6387e-5)' ;
      |         case 'Cubic Feet'
      |             name2 = 'ft^3' ;
      |             fcn2  = '/.02831685' ;
